simulink library "ammclib_bam_S32K3xx"  (R2016a)
(part 18 of 50)

      |   s16PropGainShift=ceil(log2(abs(fwkpf)));
      |   if s16PropGainShift<-31
      |     s16PropGainShift=-31;
      |   end
      |   if s16PropGainShift>31
      |     s16PropGainShift=31;
      |     warning(['Parameter s16PropGainShift of ' gcb ' exceeds the fixed-point range.']);
      |   end
      |   f32PropGain=round(fwkpf*2^(-s16PropGainShift)*2^31);
      |   if f32PropGain>2^31-1
      |     f32PropGain=2^31-1;
      |     warning(['Parameter f32PropGain of ' gcb ' exceeds the fixed-point range.']);
      |   end
      |   if f32PropGain<-2^31
      |     f32PropGain=-2^31;
      |     warning(['Parameter f32PropGain of ' gcb ' exceeds the fixed-point range.']);
      |   end
      |   s16IntegGainShift=ceil(log2(abs(kif)));
      |   if s16IntegGainShift<-31
      |     s16IntegGainShift=-31;
      |   end
      |   if s16IntegGainShift>31
      |     s16IntegGainShift=31;
      |     warning(['Parameter s16IntegGainShift of ' gcb ' exceeds the fixed-point range.']);
      |   end
      |   f32IntegGain=round(kif*2^(-s16IntegGainShift)*2^31);
      |   if f32IntegGain>2^31-1
      |     f32IntegGain=2^31-1;
      |     warning(['Parameter f32IntegGain of ' gcb ' exceeds the fixed-point range.']);
      |   end
      |   if f32IntegGain<-2^31
      |     f32IntegGain=-2^31;
      |     warning(['Parameter f32IntegGain of ' gcb ' exceeds the fixed-point range.']);
      |   end
      |   if (Idmax<0)
      |     iratio=abs(Idmax)/iscale;
      |     lowlim=0.3183098861837907*acos(iratio)-0.5;
      |   else
      |     lowlim=0.0;
      |   end
      |   f32LowerLimit=round(lowlim*2^31);
      |   if f32LowerLimit>2^31-1
      |     f32LowerLimit=2^31-1;
      |     warning(['Parameter f32LowerLimit of ' gcb ' exceeds the fixed-point range.']);
      |   end
      |   if f32LowerLimit<-2^31
      |     f32LowerLimit=-2^31;
      |     warning(['Parameter f32LowerLimit of ' gcb ' exceeds the fixed-point range.']);
      |   end
      |   f32UpperLimit=0;
      |   u16NSamples=round(log2(1.0/abs(lambdaFW)));
      |   if u16NSamples>31
      |     u16NSamples=31;
      |   end
      |   if u16NSamples<0
      |     u16NSamples=0;
      |   end
      |   if isnan(u16NSamples)
      |     if ~strcmp(u16NSamples_bkup,'0')
      |       set_param(gcb,'u16NSamples','0');
      |     end
      |   else
      |     tmps=num2str(u16NSamples);
      |     if ~strcmp(u16NSamples_bkup,tmps)
      |       set_param(gcb,'u16NSamples',tmps);
      |     end
      |   end
      |   if isnan(f32PropGain)
      |     if ~strcmp(f32PropGain_bkup,'0')
      |       set_param(gcb,'f32PropGain','0');
      |     end
      |   else
      |     tmps=num2str(f32PropGain);
      |     if ~strcmp(f32PropGain_bkup,tmps)
      |       set_param(gcb,'f32PropGain',tmps);
      |     end
      |   end
      |   if isnan(f32IntegGain)
      |     if ~strcmp(f32IntegGain_bkup,'0')
      |       set_param(gcb,'f32IntegGain','0');
      |     end
      |   else
      |     tmps=num2str(f32IntegGain);
      |     if ~strcmp(f32IntegGain_bkup,tmps)
      |       set_param(gcb,'f32IntegGain',tmps);
      |     end
      |   end
      |   if isnan(s16PropGainShift)
      |     if ~strcmp(s16PropGainShift_bkup,'0')
      |       set_param(gcb,'s16PropGainShift','0');
      |     end
      |   else
      |     tmps=num2str(s16PropGainShift);
      |     if ~strcmp(s16PropGainShift_bkup,tmps)
      |       set_param(gcb,'s16PropGainShift',tmps);
      |     end
      |   end
      |   if isnan(s16IntegGainShift)
      |     if ~strcmp(s16IntegGainShift_bkup,'0')
      |       set_param(gcb,'s16IntegGainShift','0');
      |     end
      |   else
      |     tmps=num2str(s16IntegGainShift);
      |     if ~strcmp(s16IntegGainShift_bkup,tmps)
      |       set_param(gcb,'s16IntegGainShift',tmps);
      |     end
      |   end
      |   if isnan(f32LowerLimit)
      |     if ~strcmp(f32LowerLimit_bkup,'0')
      |       set_param(gcb,'f32LowerLimit','0');
      |     end
      |   else
      |     tmps=num2str(f32LowerLimit);
      |     if ~strcmp(f32LowerLimit_bkup,tmps)
      |       set_param(gcb,'f32LowerLimit',tmps);
      |     end
      |   end
      |   if isnan(f32UpperLimit)
      |     if ~strcmp(f32UpperLimit_bkup,'0')
      |       set_param(gcb,'f32UpperLimit','0');
      |     end
      |   else
      |     tmps=num2str(f32UpperLimit);
      |     if ~strcmp(f32UpperLimit_bkup,tmps)
      |       set_param(gcb,'f32UpperLimit',tmps);
      |     end
      |   end
      | end
      mask Callback polepairs:
      | autoCalcEn=get_param(gcb,'autoCalcEn');
      | if strcmp(autoCalcEn,'on')
      |   SampleTime=Simulink.data.evalinGlobal(bdroot,get_param(gcb,'SampleTime'));
      |   if (SampleTime==-1)
      |     SampleTime=str2double(get_param(gcb,'SampleTime_1'));
      |   end
      |   u16NSamples_bkup=get_param(gcb,'u16NSamples');
      |   f32PropGain_bkup=get_param(gcb,'f32PropGain');
      |   f32IntegGain_bkup=get_param(gcb,'f32IntegGain');
      |   s16PropGainShift_bkup=get_param(gcb,'s16PropGainShift');
      |   s16IntegGainShift_bkup=get_param(gcb,'s16IntegGainShift');
      |   f32LowerLimit_bkup=get_param(gcb,'f32LowerLimit');
      |   f32UpperLimit_bkup=get_param(gcb,'f32UpperLimit');
      |   wf0=Simulink.data.evalinGlobal(bdroot,get_param(gcb,'wf0'));
      |   wksi=Simulink.data.evalinGlobal(bdroot,get_param(gcb,'wksi'));
      |   J=Simulink.data.evalinGlobal(bdroot,get_param(gcb,'J'));
      |   Kt=Simulink.data.evalinGlobal(bdroot,get_param(gcb,'Kt'));
      |   lambdaFW=Simulink.data.evalinGlobal(bdroot,get_param(gcb,'lambdaFW'));
      |   Idmax=Simulink.data.evalinGlobal(bdroot,get_param(gcb,'Idmax'));
      |   mechspeed=Simulink.data.evalinGlobal(bdroot,get_param(gcb,'mechspeed'));
      |   polepairs=Simulink.data.evalinGlobal(bdroot,get_param(gcb,'polepairs'));
      |   uscale=Simulink.data.evalinGlobal(bdroot,get_param(gcb,'uscale'));
      |   iscale=Simulink.data.evalinGlobal(bdroot,get_param(gcb,'iscale'));
      |   if (wf0<=0)
      |     warning('Natural frequency f0 must be positive.');
      |   end
      |   if (wksi<=0)
      |     warning('Current loop attenuation must be positive.');
      |   end
      |   if (wksi>1)
      |     warning('Current loop attenuation must not exceed 1.');
      |   end
      |   if (J<=0)
      |     warning('Moment of inertia J must be positive.');
      |   end
      |   if (Kt<=0)
      |     warning('Torque constant Kt must be positive.');
      |   end
      |   if (lambdaFW<0)
      |     warning('MA filter smoothing factor must be in the range 0..1.');
      |   end
      |   if (lambdaFW>1)
      |     warning('MA filter smoothing factor must be in the range 0..1.');
      |   end
      |   if (mechspeed<=0)
      |     warning('Max. speed must be positive.');
      |   end
      |   if (polepairs<1)
      |     warning('Number of pole pairs must be a natural number (1, 2, 3, ...).');
      |   end
      |   if (round(polepairs)~=polepairs)
      |     warning('Number of pole pairs must be a natural number (1, 2, 3, ...).');
      |   end
      |   if (uscale<=0)
      |     warning('U_max must be positive.');
      |   end
      |   if (iscale<=0)
      |     warning('I_max must be positive.');
      |   end
      |   w0=6.283185307179586*wf0;
      |   pgain=2.0*wksi*w0*J/Kt;
      |   igain=w0*w0*J/Kt;
      |   wmax=polepairs*mechspeed*0.1047197551196598;
      |   kif=igain*SampleTime*0.5*wmax/iscale;
      |   fwkpf=0.9*pgain*wmax/iscale;
      |   s16PropGainShift=ceil(log2(abs(fwkpf)));
      |   if s16PropGainShift<-31
      |     s16PropGainShift=-31;
      |   end
      |   if s16PropGainShift>31
      |     s16PropGainShift=31;
      |     warning(['Parameter s16PropGainShift of ' gcb ' exceeds the fixed-point range.']);
      |   end
      |   f32PropGain=round(fwkpf*2^(-s16PropGainShift)*2^31);
      |   if f32PropGain>2^31-1
      |     f32PropGain=2^31-1;
      |     warning(['Parameter f32PropGain of ' gcb ' exceeds the fixed-point range.']);
      |   end
      |   if f32PropGain<-2^31
      |     f32PropGain=-2^31;
      |     warning(['Parameter f32PropGain of ' gcb ' exceeds the fixed-point range.']);
      |   end
      |   s16IntegGainShift=ceil(log2(abs(kif)));
      |   if s16IntegGainShift<-31
      |     s16IntegGainShift=-31;
      |   end
      |   if s16IntegGainShift>31
      |     s16IntegGainShift=31;
      |     warning(['Parameter s16IntegGainShift of ' gcb ' exceeds the fixed-point range.']);
      |   end
      |   f32IntegGain=round(kif*2^(-s16IntegGainShift)*2^31);
      |   if f32IntegGain>2^31-1
      |     f32IntegGain=2^31-1;
      |     warning(['Parameter f32IntegGain of ' gcb ' exceeds the fixed-point range.']);
      |   end
      |   if f32IntegGain<-2^31
      |     f32IntegGain=-2^31;
      |     warning(['Parameter f32IntegGain of ' gcb ' exceeds the fixed-point range.']);
      |   end
      |   if (Idmax<0)
      |     iratio=abs(Idmax)/iscale;
      |     lowlim=0.3183098861837907*acos(iratio)-0.5;
      |   else
      |     lowlim=0.0;
      |   end
      |   f32LowerLimit=round(lowlim*2^31);
      |   if f32LowerLimit>2^31-1
      |     f32LowerLimit=2^31-1;
      |     warning(['Parameter f32LowerLimit of ' gcb ' exceeds the fixed-point range.']);
      |   end
      |   if f32LowerLimit<-2^31
      |     f32LowerLimit=-2^31;
      |     warning(['Parameter f32LowerLimit of ' gcb ' exceeds the fixed-point range.']);
      |   end
      |   f32UpperLimit=0;
      |   u16NSamples=round(log2(1.0/abs(lambdaFW)));
      |   if u16NSamples>31
      |     u16NSamples=31;
      |   end
      |   if u16NSamples<0
      |     u16NSamples=0;
      |   end
      |   if isnan(u16NSamples)
      |     if ~strcmp(u16NSamples_bkup,'0')
      |       set_param(gcb,'u16NSamples','0');
      |     end
      |   else
      |     tmps=num2str(u16NSamples);
      |     if ~strcmp(u16NSamples_bkup,tmps)
      |       set_param(gcb,'u16NSamples',tmps);
      |     end
      |   end
      |   if isnan(f32PropGain)
      |     if ~strcmp(f32PropGain_bkup,'0')
      |       set_param(gcb,'f32PropGain','0');
      |     end
      |   else
      |     tmps=num2str(f32PropGain);
      |     if ~strcmp(f32PropGain_bkup,tmps)
      |       set_param(gcb,'f32PropGain',tmps);
      |     end
      |   end
      |   if isnan(f32IntegGain)
      |     if ~strcmp(f32IntegGain_bkup,'0')
      |       set_param(gcb,'f32IntegGain','0');
      |     end
      |   else
      |     tmps=num2str(f32IntegGain);
      |     if ~strcmp(f32IntegGain_bkup,tmps)
      |       set_param(gcb,'f32IntegGain',tmps);
      |     end
      |   end
      |   if isnan(s16PropGainShift)
      |     if ~strcmp(s16PropGainShift_bkup,'0')
      |       set_param(gcb,'s16PropGainShift','0');
      |     end
      |   else
      |     tmps=num2str(s16PropGainShift);
      |     if ~strcmp(s16PropGainShift_bkup,tmps)
      |       set_param(gcb,'s16PropGainShift',tmps);
      |     end
      |   end
      |   if isnan(s16IntegGainShift)
      |     if ~strcmp(s16IntegGainShift_bkup,'0')
      |       set_param(gcb,'s16IntegGainShift','0');
      |     end
      |   else
      |     tmps=num2str(s16IntegGainShift);
      |     if ~strcmp(s16IntegGainShift_bkup,tmps)
      |       set_param(gcb,'s16IntegGainShift',tmps);
      |     end
      |   end
      |   if isnan(f32LowerLimit)
      |     if ~strcmp(f32LowerLimit_bkup,'0')
      |       set_param(gcb,'f32LowerLimit','0');
      |     end
      |   else
      |     tmps=num2str(f32LowerLimit);
      |     if ~strcmp(f32LowerLimit_bkup,tmps)
      |       set_param(gcb,'f32LowerLimit',tmps);
      |     end
      |   end
      |   if isnan(f32UpperLimit)
      |     if ~strcmp(f32UpperLimit_bkup,'0')
      |       set_param(gcb,'f32UpperLimit','0');
      |     end
      |   else
      |     tmps=num2str(f32UpperLimit);
      |     if ~strcmp(f32UpperLimit_bkup,tmps)
      |       set_param(gcb,'f32UpperLimit',tmps);
      |     end
      |   end
      | end
      mask Callback uscale:
      | autoCalcEn=get_param(gcb,'autoCalcEn');
      | if strcmp(autoCalcEn,'on')
      |   SampleTime=Simulink.data.evalinGlobal(bdroot,get_param(gcb,'SampleTime'));
      |   if (SampleTime==-1)
      |     SampleTime=str2double(get_param(gcb,'SampleTime_1'));
      |   end
      |   u16NSamples_bkup=get_param(gcb,'u16NSamples');
      |   f32PropGain_bkup=get_param(gcb,'f32PropGain');
      |   f32IntegGain_bkup=get_param(gcb,'f32IntegGain');
      |   s16PropGainShift_bkup=get_param(gcb,'s16PropGainShift');
      |   s16IntegGainShift_bkup=get_param(gcb,'s16IntegGainShift');
      |   f32LowerLimit_bkup=get_param(gcb,'f32LowerLimit');
      |   f32UpperLimit_bkup=get_param(gcb,'f32UpperLimit');
      |   wf0=Simulink.data.evalinGlobal(bdroot,get_param(gcb,'wf0'));
      |   wksi=Simulink.data.evalinGlobal(bdroot,get_param(gcb,'wksi'));
      |   J=Simulink.data.evalinGlobal(bdroot,get_param(gcb,'J'));
      |   Kt=Simulink.data.evalinGlobal(bdroot,get_param(gcb,'Kt'));
      |   lambdaFW=Simulink.data.evalinGlobal(bdroot,get_param(gcb,'lambdaFW'));
      |   Idmax=Simulink.data.evalinGlobal(bdroot,get_param(gcb,'Idmax'));
      |   mechspeed=Simulink.data.evalinGlobal(bdroot,get_param(gcb,'mechspeed'));
      |   polepairs=Simulink.data.evalinGlobal(bdroot,get_param(gcb,'polepairs'));
      |   uscale=Simulink.data.evalinGlobal(bdroot,get_param(gcb,'uscale'));
      |   iscale=Simulink.data.evalinGlobal(bdroot,get_param(gcb,'iscale'));
      |   if (wf0<=0)
      |     warning('Natural frequency f0 must be positive.');
      |   end
      |   if (wksi<=0)
      |     warning('Current loop attenuation must be positive.');
      |   end
      |   if (wksi>1)
      |     warning('Current loop attenuation must not exceed 1.');
      |   end
      |   if (J<=0)
      |     warning('Moment of inertia J must be positive.');
      |   end
      |   if (Kt<=0)
      |     warning('Torque constant Kt must be positive.');
      |   end
      |   if (lambdaFW<0)
      |     warning('MA filter smoothing factor must be in the range 0..1.');
      |   end
      |   if (lambdaFW>1)
      |     warning('MA filter smoothing factor must be in the range 0..1.');
      |   end
      |   if (mechspeed<=0)
      |     warning('Max. speed must be positive.');
      |   end
      |   if (polepairs<1)
      |     warning('Number of pole pairs must be a natural number (1, 2, 3, ...).');
      |   end
      |   if (round(polepairs)~=polepairs)
      |     warning('Number of pole pairs must be a natural number (1, 2, 3, ...).');
      |   end
      |   if (uscale<=0)
      |     warning('U_max must be positive.');
      |   end
      |   if (iscale<=0)
      |     warning('I_max must be positive.');
      |   end
      |   w0=6.283185307179586*wf0;
      |   pgain=2.0*wksi*w0*J/Kt;
      |   igain=w0*w0*J/Kt;
      |   wmax=polepairs*mechspeed*0.1047197551196598;
      |   kif=igain*SampleTime*0.5*wmax/iscale;
      |   fwkpf=0.9*pgain*wmax/iscale;
      |   s16PropGainShift=ceil(log2(abs(fwkpf)));
      |   if s16PropGainShift<-31
      |     s16PropGainShift=-31;
      |   end
      |   if s16PropGainShift>31
      |     s16PropGainShift=31;
      |     warning(['Parameter s16PropGainShift of ' gcb ' exceeds the fixed-point range.']);
      |   end
      |   f32PropGain=round(fwkpf*2^(-s16PropGainShift)*2^31);
      |   if f32PropGain>2^31-1
      |     f32PropGain=2^31-1;
      |     warning(['Parameter f32PropGain of ' gcb ' exceeds the fixed-point range.']);
      |   end
      |   if f32PropGain<-2^31
      |     f32PropGain=-2^31;
      |     warning(['Parameter f32PropGain of ' gcb ' exceeds the fixed-point range.']);
      |   end
      |   s16IntegGainShift=ceil(log2(abs(kif)));
      |   if s16IntegGainShift<-31
      |     s16IntegGainShift=-31;
      |   end
      |   if s16IntegGainShift>31
      |     s16IntegGainShift=31;
      |     warning(['Parameter s16IntegGainShift of ' gcb ' exceeds the fixed-point range.']);
      |   end
      |   f32IntegGain=round(kif*2^(-s16IntegGainShift)*2^31);
      |   if f32IntegGain>2^31-1
      |     f32IntegGain=2^31-1;
      |     warning(['Parameter f32IntegGain of ' gcb ' exceeds the fixed-point range.']);
      |   end
      |   if f32IntegGain<-2^31
      |     f32IntegGain=-2^31;
      |     warning(['Parameter f32IntegGain of ' gcb ' exceeds the fixed-point range.']);
      |   end
      |   if (Idmax<0)
      |     iratio=abs(Idmax)/iscale;
      |     lowlim=0.3183098861837907*acos(iratio)-0.5;
      |   else
      |     lowlim=0.0;
      |   end
      |   f32LowerLimit=round(lowlim*2^31);
      |   if f32LowerLimit>2^31-1
      |     f32LowerLimit=2^31-1;
      |     warning(['Parameter f32LowerLimit of ' gcb ' exceeds the fixed-point range.']);
      |   end
      |   if f32LowerLimit<-2^31
      |     f32LowerLimit=-2^31;
      |     warning(['Parameter f32LowerLimit of ' gcb ' exceeds the fixed-point range.']);
      |   end
      |   f32UpperLimit=0;
      |   u16NSamples=round(log2(1.0/abs(lambdaFW)));
      |   if u16NSamples>31
      |     u16NSamples=31;
      |   end
      |   if u16NSamples<0
      |     u16NSamples=0;
      |   end
      |   if isnan(u16NSamples)
      |     if ~strcmp(u16NSamples_bkup,'0')
      |       set_param(gcb,'u16NSamples','0');
      |     end
      |   else
      |     tmps=num2str(u16NSamples);
      |     if ~strcmp(u16NSamples_bkup,tmps)
      |       set_param(gcb,'u16NSamples',tmps);
      |     end
      |   end
      |   if isnan(f32PropGain)
      |     if ~strcmp(f32PropGain_bkup,'0')
      |       set_param(gcb,'f32PropGain','0');
      |     end
      |   else
      |     tmps=num2str(f32PropGain);
      |     if ~strcmp(f32PropGain_bkup,tmps)
      |       set_param(gcb,'f32PropGain',tmps);
      |     end
      |   end
      |   if isnan(f32IntegGain)
      |     if ~strcmp(f32IntegGain_bkup,'0')
      |       set_param(gcb,'f32IntegGain','0');
      |     end
      |   else
      |     tmps=num2str(f32IntegGain);
      |     if ~strcmp(f32IntegGain_bkup,tmps)
      |       set_param(gcb,'f32IntegGain',tmps);
      |     end
      |   end
      |   if isnan(s16PropGainShift)
      |     if ~strcmp(s16PropGainShift_bkup,'0')
      |       set_param(gcb,'s16PropGainShift','0');
      |     end
      |   else
      |     tmps=num2str(s16PropGainShift);
      |     if ~strcmp(s16PropGainShift_bkup,tmps)
      |       set_param(gcb,'s16PropGainShift',tmps);
      |     end
      |   end
      |   if isnan(s16IntegGainShift)
      |     if ~strcmp(s16IntegGainShift_bkup,'0')
      |       set_param(gcb,'s16IntegGainShift','0');
      |     end
      |   else
      |     tmps=num2str(s16IntegGainShift);
      |     if ~strcmp(s16IntegGainShift_bkup,tmps)
      |       set_param(gcb,'s16IntegGainShift',tmps);
      |     end
      |   end
      |   if isnan(f32LowerLimit)
      |     if ~strcmp(f32LowerLimit_bkup,'0')
      |       set_param(gcb,'f32LowerLimit','0');
      |     end
      |   else
      |     tmps=num2str(f32LowerLimit);
      |     if ~strcmp(f32LowerLimit_bkup,tmps)
      |       set_param(gcb,'f32LowerLimit',tmps);
      |     end
      |   end
      |   if isnan(f32UpperLimit)
      |     if ~strcmp(f32UpperLimit_bkup,'0')
      |       set_param(gcb,'f32UpperLimit','0');
      |     end
      |   else
      |     tmps=num2str(f32UpperLimit);
      |     if ~strcmp(f32UpperLimit_bkup,tmps)
      |       set_param(gcb,'f32UpperLimit',tmps);
      |     end
      |   end
      | end
      mask Callback iscale:
      | autoCalcEn=get_param(gcb,'autoCalcEn');
      | if strcmp(autoCalcEn,'on')
      |   SampleTime=Simulink.data.evalinGlobal(bdroot,get_param(gcb,'SampleTime'));
      |   if (SampleTime==-1)
      |     SampleTime=str2double(get_param(gcb,'SampleTime_1'));
      |   end
      |   u16NSamples_bkup=get_param(gcb,'u16NSamples');
      |   f32PropGain_bkup=get_param(gcb,'f32PropGain');
      |   f32IntegGain_bkup=get_param(gcb,'f32IntegGain');
      |   s16PropGainShift_bkup=get_param(gcb,'s16PropGainShift');
      |   s16IntegGainShift_bkup=get_param(gcb,'s16IntegGainShift');
      |   f32LowerLimit_bkup=get_param(gcb,'f32LowerLimit');
      |   f32UpperLimit_bkup=get_param(gcb,'f32UpperLimit');
      |   wf0=Simulink.data.evalinGlobal(bdroot,get_param(gcb,'wf0'));
      |   wksi=Simulink.data.evalinGlobal(bdroot,get_param(gcb,'wksi'));
      |   J=Simulink.data.evalinGlobal(bdroot,get_param(gcb,'J'));
      |   Kt=Simulink.data.evalinGlobal(bdroot,get_param(gcb,'Kt'));
      |   lambdaFW=Simulink.data.evalinGlobal(bdroot,get_param(gcb,'lambdaFW'));
      |   Idmax=Simulink.data.evalinGlobal(bdroot,get_param(gcb,'Idmax'));
      |   mechspeed=Simulink.data.evalinGlobal(bdroot,get_param(gcb,'mechspeed'));
      |   polepairs=Simulink.data.evalinGlobal(bdroot,get_param(gcb,'polepairs'));
      |   uscale=Simulink.data.evalinGlobal(bdroot,get_param(gcb,'uscale'));
      |   iscale=Simulink.data.evalinGlobal(bdroot,get_param(gcb,'iscale'));
      |   if (wf0<=0)
      |     warning('Natural frequency f0 must be positive.');
      |   end
      |   if (wksi<=0)
      |     warning('Current loop attenuation must be positive.');
      |   end
      |   if (wksi>1)
      |     warning('Current loop attenuation must not exceed 1.');
      |   end
      |   if (J<=0)
      |     warning('Moment of inertia J must be positive.');
      |   end
      |   if (Kt<=0)
      |     warning('Torque constant Kt must be positive.');
      |   end
      |   if (lambdaFW<0)
      |     warning('MA filter smoothing factor must be in the range 0..1.');
      |   end
      |   if (lambdaFW>1)
      |     warning('MA filter smoothing factor must be in the range 0..1.');
      |   end
      |   if (mechspeed<=0)
      |     warning('Max. speed must be positive.');
      |   end
      |   if (polepairs<1)
      |     warning('Number of pole pairs must be a natural number (1, 2, 3, ...).');
      |   end
      |   if (round(polepairs)~=polepairs)
      |     warning('Number of pole pairs must be a natural number (1, 2, 3, ...).');
      |   end
      |   if (uscale<=0)
      |     warning('U_max must be positive.');
      |   end
      |   if (iscale<=0)
      |     warning('I_max must be positive.');
      |   end
      |   w0=6.283185307179586*wf0;
      |   pgain=2.0*wksi*w0*J/Kt;
      |   igain=w0*w0*J/Kt;
      |   wmax=polepairs*mechspeed*0.1047197551196598;
      |   kif=igain*SampleTime*0.5*wmax/iscale;
      |   fwkpf=0.9*pgain*wmax/iscale;
      |   s16PropGainShift=ceil(log2(abs(fwkpf)));
      |   if s16PropGainShift<-31
      |     s16PropGainShift=-31;
      |   end
      |   if s16PropGainShift>31
      |     s16PropGainShift=31;
      |     warning(['Parameter s16PropGainShift of ' gcb ' exceeds the fixed-point range.']);
      |   end
      |   f32PropGain=round(fwkpf*2^(-s16PropGainShift)*2^31);
      |   if f32PropGain>2^31-1
      |     f32PropGain=2^31-1;
      |     warning(['Parameter f32PropGain of ' gcb ' exceeds the fixed-point range.']);
      |   end
      |   if f32PropGain<-2^31
      |     f32PropGain=-2^31;
      |     warning(['Parameter f32PropGain of ' gcb ' exceeds the fixed-point range.']);
      |   end
      |   s16IntegGainShift=ceil(log2(abs(kif)));
      |   if s16IntegGainShift<-31
      |     s16IntegGainShift=-31;
      |   end
      |   if s16IntegGainShift>31
      |     s16IntegGainShift=31;
      |     warning(['Parameter s16IntegGainShift of ' gcb ' exceeds the fixed-point range.']);
      |   end
      |   f32IntegGain=round(kif*2^(-s16IntegGainShift)*2^31);
      |   if f32IntegGain>2^31-1
      |     f32IntegGain=2^31-1;
      |     warning(['Parameter f32IntegGain of ' gcb ' exceeds the fixed-point range.']);
      |   end
      |   if f32IntegGain<-2^31
      |     f32IntegGain=-2^31;
      |     warning(['Parameter f32IntegGain of ' gcb ' exceeds the fixed-point range.']);
      |   end
      |   if (Idmax<0)
      |     iratio=abs(Idmax)/iscale;
      |     lowlim=0.3183098861837907*acos(iratio)-0.5;
      |   else
      |     lowlim=0.0;
      |   end
      |   f32LowerLimit=round(lowlim*2^31);
      |   if f32LowerLimit>2^31-1
      |     f32LowerLimit=2^31-1;
      |     warning(['Parameter f32LowerLimit of ' gcb ' exceeds the fixed-point range.']);
      |   end
      |   if f32LowerLimit<-2^31
      |     f32LowerLimit=-2^31;
      |     warning(['Parameter f32LowerLimit of ' gcb ' exceeds the fixed-point range.']);
      |   end
      |   f32UpperLimit=0;
      |   u16NSamples=round(log2(1.0/abs(lambdaFW)));
      |   if u16NSamples>31
      |     u16NSamples=31;
      |   end
      |   if u16NSamples<0
      |     u16NSamples=0;
      |   end
      |   if isnan(u16NSamples)
      |     if ~strcmp(u16NSamples_bkup,'0')
      |       set_param(gcb,'u16NSamples','0');
      |     end
      |   else
      |     tmps=num2str(u16NSamples);
      |     if ~strcmp(u16NSamples_bkup,tmps)
      |       set_param(gcb,'u16NSamples',tmps);
      |     end
      |   end
      |   if isnan(f32PropGain)
      |     if ~strcmp(f32PropGain_bkup,'0')
      |       set_param(gcb,'f32PropGain','0');
      |     end
      |   else
      |     tmps=num2str(f32PropGain);
      |     if ~strcmp(f32PropGain_bkup,tmps)
      |       set_param(gcb,'f32PropGain',tmps);
      |     end
      |   end
      |   if isnan(f32IntegGain)
      |     if ~strcmp(f32IntegGain_bkup,'0')
      |       set_param(gcb,'f32IntegGain','0');
      |     end
      |   else
      |     tmps=num2str(f32IntegGain);
      |     if ~strcmp(f32IntegGain_bkup,tmps)
      |       set_param(gcb,'f32IntegGain',tmps);
      |     end
      |   end
      |   if isnan(s16PropGainShift)
      |     if ~strcmp(s16PropGainShift_bkup,'0')
      |       set_param(gcb,'s16PropGainShift','0');
      |     end
      |   else
      |     tmps=num2str(s16PropGainShift);
      |     if ~strcmp(s16PropGainShift_bkup,tmps)
      |       set_param(gcb,'s16PropGainShift',tmps);
      |     end
      |   end
      |   if isnan(s16IntegGainShift)
      |     if ~strcmp(s16IntegGainShift_bkup,'0')
      |       set_param(gcb,'s16IntegGainShift','0');
      |     end
      |   else
      |     tmps=num2str(s16IntegGainShift);
      |     if ~strcmp(s16IntegGainShift_bkup,tmps)
      |       set_param(gcb,'s16IntegGainShift',tmps);
      |     end
      |   end
      |   if isnan(f32LowerLimit)
      |     if ~strcmp(f32LowerLimit_bkup,'0')
      |       set_param(gcb,'f32LowerLimit','0');
      |     end
      |   else
      |     tmps=num2str(f32LowerLimit);
      |     if ~strcmp(f32LowerLimit_bkup,tmps)
      |       set_param(gcb,'f32LowerLimit',tmps);
      |     end
      |   end
      |   if isnan(f32UpperLimit)
      |     if ~strcmp(f32UpperLimit_bkup,'0')
      |       set_param(gcb,'f32UpperLimit','0');
      |     end
      |   else
      |     tmps=num2str(f32UpperLimit);
      |     if ~strcmp(f32UpperLimit_bkup,tmps)
      |       set_param(gcb,'f32UpperLimit',tmps);
      |     end
      |   end
      | end
      mask Callback autoCalcEn:
      | maskStr=get_param(gcb,'showStates');
      | if strcmp(maskStr,'Hide (faster execution)')
      |   p=Simulink.Mask.get(gcb);
      |   autoCalcEn=get_param(gcb,'autoCalcEn');
      |   hintText=p.getDialogControl('timeHint');
      |   if strcmp(autoCalcEn,'on')
      |     param=p.getParameter('iscale');
      |     if strcmp(param.Enabled,'off')
      |       SampleTime=Simulink.data.evalinGlobal(bdroot,get_param(gcb,'SampleTime'));
      |       if SampleTime==-1
      |         SampleTime=str2double(get_param(gcb,'SampleTime_1'));
      |         if isnan(SampleTime)
      |           hintText.Prompt=['Note: Implementation parameters cannot be calculated yet because the block''s inherited sample time is unknown. Simulink will update the sample time when you run the simulation.'];
      |         else
      |           hintText.Prompt=['Caution: Implementation parameters depend on inherited sample time. Make sure that the sample time of the block''s inputs corresponds to the sampling period in the target application.'];
      |         end
      |       else
      |         hintText.Prompt='Caution: Implementation parameters depend on the sample time. Make sure that the simulation time step corresponds to the sampling period in the target application.';
      |       end
      |       p=Simulink.Mask.get(gcb);
      |       param=p.getParameter('wf0');
      |       param.set('Enabled','on');
      |       param=p.getParameter('wksi');
      |       param.set('Enabled','on');
      |       param=p.getParameter('J');
      |       param.set('Enabled','on');
      |       param=p.getParameter('Kt');
      |       param.set('Enabled','on');
      |       param=p.getParameter('lambdaFW');
      |       param.set('Enabled','on');
      |       param=p.getParameter('Idmax');
      |       param.set('Enabled','on');
      |       param=p.getParameter('mechspeed');
      |       param.set('Enabled','on');
      |       param=p.getParameter('polepairs');
      |       param.set('Enabled','on');
      |       param=p.getParameter('uscale');
      |       param.set('Enabled','on');
      |       param=p.getParameter('iscale');
      |       param.set('Enabled','on');
      |     else
      |       SampleTime=Simulink.data.evalinGlobal(bdroot,get_param(gcb,'SampleTime'));
      |       if SampleTime==-1
      |         SampleTime=str2double(get_param(gcb,'SampleTime_1'));
      |       end
      |     end
      |     u16NSamples_bkup=get_param(gcb,'u16NSamples');
      |     f32PropGain_bkup=get_param(gcb,'f32PropGain');
      |     f32IntegGain_bkup=get_param(gcb,'f32IntegGain');
      |     s16PropGainShift_bkup=get_param(gcb,'s16PropGainShift');
      |     s16IntegGainShift_bkup=get_param(gcb,'s16IntegGainShift');
      |     f32LowerLimit_bkup=get_param(gcb,'f32LowerLimit');
      |     f32UpperLimit_bkup=get_param(gcb,'f32UpperLimit');
      |     wf0=Simulink.data.evalinGlobal(bdroot,get_param(gcb,'wf0'));
      |     wksi=Simulink.data.evalinGlobal(bdroot,get_param(gcb,'wksi'));
      |     J=Simulink.data.evalinGlobal(bdroot,get_param(gcb,'J'));
      |     Kt=Simulink.data.evalinGlobal(bdroot,get_param(gcb,'Kt'));
      |     lambdaFW=Simulink.data.evalinGlobal(bdroot,get_param(gcb,'lambdaFW'));
      |     Idmax=Simulink.data.evalinGlobal(bdroot,get_param(gcb,'Idmax'));
      |     mechspeed=Simulink.data.evalinGlobal(bdroot,get_param(gcb,'mechspeed'));
      |     polepairs=Simulink.data.evalinGlobal(bdroot,get_param(gcb,'polepairs'));
      |     uscale=Simulink.data.evalinGlobal(bdroot,get_param(gcb,'uscale'));
      |     iscale=Simulink.data.evalinGlobal(bdroot,get_param(gcb,'iscale'));
      |     if (wf0<=0)
      |       warning('Natural frequency f0 must be positive.');
      |     end
      |     if (wksi<=0)
      |       warning('Current loop attenuation must be positive.');
      |     end
      |     if (wksi>1)
      |       warning('Current loop attenuation must not exceed 1.');
      |     end
      |     if (J<=0)
      |       warning('Moment of inertia J must be positive.');
      |     end
      |     if (Kt<=0)
      |       warning('Torque constant Kt must be positive.');
      |     end
      |     if (lambdaFW<0)
      |       warning('MA filter smoothing factor must be in the range 0..1.');
      |     end
      |     if (lambdaFW>1)
      |       warning('MA filter smoothing factor must be in the range 0..1.');
      |     end
      |     if (mechspeed<=0)
      |       warning('Max. speed must be positive.');
      |     end
      |     if (polepairs<1)
      |       warning('Number of pole pairs must be a natural number (1, 2, 3, ...).');
      |     end
      |     if (round(polepairs)~=polepairs)
      |       warning('Number of pole pairs must be a natural number (1, 2, 3, ...).');
      |     end
      |     if (uscale<=0)
      |       warning('U_max must be positive.');
      |     end
      |     if (iscale<=0)
      |       warning('I_max must be positive.');
      |     end
      |     w0=6.283185307179586*wf0;
      |     pgain=2.0*wksi*w0*J/Kt;
      |     igain=w0*w0*J/Kt;
      |     wmax=polepairs*mechspeed*0.1047197551196598;
      |     kif=igain*SampleTime*0.5*wmax/iscale;
      |     fwkpf=0.9*pgain*wmax/iscale;
      |     s16PropGainShift=ceil(log2(abs(fwkpf)));
      |     if s16PropGainShift<-31
      |       s16PropGainShift=-31;
      |     end
      |     if s16PropGainShift>31
      |       s16PropGainShift=31;
      |       warning(['Parameter s16PropGainShift of ' gcb ' exceeds the fixed-point range.']);
      |     end
      |     f32PropGain=round(fwkpf*2^(-s16PropGainShift)*2^31);
      |     if f32PropGain>2^31-1
      |       f32PropGain=2^31-1;
      |       warning(['Parameter f32PropGain of ' gcb ' exceeds the fixed-point range.']);
      |     end
      |     if f32PropGain<-2^31
      |       f32PropGain=-2^31;
      |       warning(['Parameter f32PropGain of ' gcb ' exceeds the fixed-point range.']);
      |     end
      |     s16IntegGainShift=ceil(log2(abs(kif)));
      |     if s16IntegGainShift<-31
      |       s16IntegGainShift=-31;
      |     end
      |     if s16IntegGainShift>31
      |       s16IntegGainShift=31;
      |       warning(['Parameter s16IntegGainShift of ' gcb ' exceeds the fixed-point range.']);
      |     end
      |     f32IntegGain=round(kif*2^(-s16IntegGainShift)*2^31);
      |     if f32IntegGain>2^31-1
      |       f32IntegGain=2^31-1;
      |       warning(['Parameter f32IntegGain of ' gcb ' exceeds the fixed-point range.']);
      |     end
      |     if f32IntegGain<-2^31
      |       f32IntegGain=-2^31;
      |       warning(['Parameter f32IntegGain of ' gcb ' exceeds the fixed-point range.']);
      |     end
      |     if (Idmax<0)
      |       iratio=abs(Idmax)/iscale;
      |       lowlim=0.3183098861837907*acos(iratio)-0.5;
      |     else
      |       lowlim=0.0;
      |     end
      |     f32LowerLimit=round(lowlim*2^31);
      |     if f32LowerLimit>2^31-1
      |       f32LowerLimit=2^31-1;
      |       warning(['Parameter f32LowerLimit of ' gcb ' exceeds the fixed-point range.']);
      |     end
      |     if f32LowerLimit<-2^31
      |       f32LowerLimit=-2^31;
      |       warning(['Parameter f32LowerLimit of ' gcb ' exceeds the fixed-point range.']);
      |     end
      |     f32UpperLimit=0;
      |     u16NSamples=round(log2(1.0/abs(lambdaFW)));
      |     if u16NSamples>31
      |       u16NSamples=31;
      |     end
      |     if u16NSamples<0
      |       u16NSamples=0;
      |     end
      |     if isnan(u16NSamples)
      |       if ~strcmp(u16NSamples_bkup,'0')
      |         set_param(gcb,'u16NSamples','0');
      |       end
      |     else
      |       tmps=num2str(u16NSamples);
      |       if ~strcmp(u16NSamples_bkup,tmps)
      |         set_param(gcb,'u16NSamples',tmps);
      |       end
      |     end
      |     if isnan(f32PropGain)
      |       if ~strcmp(f32PropGain_bkup,'0')
      |         set_param(gcb,'f32PropGain','0');
      |       end
      |     else
      |       tmps=num2str(f32PropGain);
      |       if ~strcmp(f32PropGain_bkup,tmps)
      |         set_param(gcb,'f32PropGain',tmps);
      |       end
      |     end
      |     if isnan(f32IntegGain)
      |       if ~strcmp(f32IntegGain_bkup,'0')
      |         set_param(gcb,'f32IntegGain','0');
      |       end
      |     else
      |       tmps=num2str(f32IntegGain);
      |       if ~strcmp(f32IntegGain_bkup,tmps)
      |         set_param(gcb,'f32IntegGain',tmps);
      |       end
      |     end
      |     if isnan(s16PropGainShift)
      |       if ~strcmp(s16PropGainShift_bkup,'0')
      |         set_param(gcb,'s16PropGainShift','0');
      |       end
      |     else
      |       tmps=num2str(s16PropGainShift);
      |       if ~strcmp(s16PropGainShift_bkup,tmps)
      |         set_param(gcb,'s16PropGainShift',tmps);
      |       end
      |     end
      |     if isnan(s16IntegGainShift)
      |       if ~strcmp(s16IntegGainShift_bkup,'0')
      |         set_param(gcb,'s16IntegGainShift','0');
      |       end
      |     else
      |       tmps=num2str(s16IntegGainShift);
      |       if ~strcmp(s16IntegGainShift_bkup,tmps)
      |         set_param(gcb,'s16IntegGainShift',tmps);
      |       end
      |     end
      |     if isnan(f32LowerLimit)
      |       if ~strcmp(f32LowerLimit_bkup,'0')
      |         set_param(gcb,'f32LowerLimit','0');
      |       end
      |     else
      |       tmps=num2str(f32LowerLimit);
      |       if ~strcmp(f32LowerLimit_bkup,tmps)
      |         set_param(gcb,'f32LowerLimit',tmps);
      |       end
      |     end
      |     if isnan(f32UpperLimit)
      |       if ~strcmp(f32UpperLimit_bkup,'0')
      |         set_param(gcb,'f32UpperLimit','0');
      |       end
      |     else
      |       tmps=num2str(f32UpperLimit);
      |       if ~strcmp(f32UpperLimit_bkup,tmps)
      |         set_param(gcb,'f32UpperLimit',tmps);
      |       end
      |     end
      |   else
      |     param=p.getParameter('iscale');
      |     if strcmp(param.Enabled,'on')
      |       hintText.Prompt='Caution: Implementation parameters are fixed.';
      |       p=Simulink.Mask.get(gcb);
      |       param=p.getParameter('wf0');
      |       param.set('Enabled','off');
      |       param=p.getParameter('wksi');
      |       param.set('Enabled','off');
      |       param=p.getParameter('J');
      |       param.set('Enabled','off');
      |       param=p.getParameter('Kt');
      |       param.set('Enabled','off');
      |       param=p.getParameter('lambdaFW');
      |       param.set('Enabled','off');
      |       param=p.getParameter('Idmax');
      |       param.set('Enabled','off');
      |       param=p.getParameter('mechspeed');
      |       param.set('Enabled','off');
      |       param=p.getParameter('polepairs');
      |       param.set('Enabled','off');
      |       param=p.getParameter('uscale');
      |       param.set('Enabled','off');
      |       param=p.getParameter('iscale');
      |       param.set('Enabled','off');
      |     end
      |   end
      | end
      mask DialogControl CompBut Prompt: Recalculate sample times
      mask DialogControl CompBut Tooltip: Simulink updates the sample times of all blocks when the simulation is run. This button will update the sample times now.
      mask DialogControl CompBut Callback:
      | btn=questdlg('This will apply all changes in all open dialog boxes and update the schematic. Do you want to proceed?','Apply all changes','Continue','Cancel','Continue');
      | if strcmp(btn,'Continue')
      |   dlgs=DAStudio.ToolRoot.getOpenDialogs;
      |   for i=1:length(dlgs)
      |     dlgs(i).apply;
      |   end
      |   try
      |     SampleTime_1=str2double(get_param(gcb,'SampleTime_1'));
      |     ts=Simulink.Block.getSampleTimes(gcb);
      |     ts=ts(1).Value(1);
      |     if (SampleTime_1 ~= ts)
      |       SampleTime_1=ts;
      |       set_param(gcb,'SampleTime_1',num2str(ts));
      |       autoCalcEn=get_param(gcb,'autoCalcEn');
      |       if strcmp(autoCalcEn,'on')
      |         SampleTime=Simulink.data.evalinGlobal(bdroot,get_param(gcb,'SampleTime'));
      |         p=Simulink.Mask.get(gcb);
      |         hintText=p.getDialogControl('timeHint');
      |         if SampleTime==-1
      |           SampleTime=SampleTime_1;
      |           hintText.Prompt='Caution: Implementation parameters depend on inherited sample time. Make sure that the sample time of the block''s inputs corresponds to the sampling period in the target application.';
      |         else
      |           hintText.Prompt='Caution: Implementation parameters depend on the sample time. Make sure that the simulation time step corresponds to the sampling period in the target application.';
      |         end
      |         u16NSamples_bkup=get_param(gcb,'u16NSamples');
      |         f32PropGain_bkup=get_param(gcb,'f32PropGain');
      |         f32IntegGain_bkup=get_param(gcb,'f32IntegGain');
      |         s16PropGainShift_bkup=get_param(gcb,'s16PropGainShift');
      |         s16IntegGainShift_bkup=get_param(gcb,'s16IntegGainShift');
      |         f32LowerLimit_bkup=get_param(gcb,'f32LowerLimit');
      |         f32UpperLimit_bkup=get_param(gcb,'f32UpperLimit');
      |         wf0=Simulink.data.evalinGlobal(bdroot,get_param(gcb,'wf0'));
      |         wksi=Simulink.data.evalinGlobal(bdroot,get_param(gcb,'wksi'));
      |         J=Simulink.data.evalinGlobal(bdroot,get_param(gcb,'J'));
      |         Kt=Simulink.data.evalinGlobal(bdroot,get_param(gcb,'Kt'));
      |         lambdaFW=Simulink.data.evalinGlobal(bdroot,get_param(gcb,'lambdaFW'));
      |         Idmax=Simulink.data.evalinGlobal(bdroot,get_param(gcb,'Idmax'));
      |         mechspeed=Simulink.data.evalinGlobal(bdroot,get_param(gcb,'mechspeed'));
      |         polepairs=Simulink.data.evalinGlobal(bdroot,get_param(gcb,'polepairs'));
      |         uscale=Simulink.data.evalinGlobal(bdroot,get_param(gcb,'uscale'));
      |         iscale=Simulink.data.evalinGlobal(bdroot,get_param(gcb,'iscale'));
      |         if (wf0<=0)
      |           warning('Natural frequency f0 must be positive.');
      |         end
      |         if (wksi<=0)
      |           warning('Current loop attenuation must be positive.');
      |         end
      |         if (wksi>1)
      |           warning('Current loop attenuation must not exceed 1.');
      |         end
      |         if (J<=0)
      |           warning('Moment of inertia J must be positive.');
      |         end
      |         if (Kt<=0)
      |           warning('Torque constant Kt must be positive.');
      |         end
      |         if (lambdaFW<0)
      |           warning('MA filter smoothing factor must be in the range 0..1.');
      |         end
      |         if (lambdaFW>1)
      |           warning('MA filter smoothing factor must be in the range 0..1.');
      |         end
      |         if (mechspeed<=0)
      |           warning('Max. speed must be positive.');
      |         end
      |         if (polepairs<1)
      |           warning('Number of pole pairs must be a natural number (1, 2, 3, ...).');
      |         end
      |         if (round(polepairs)~=polepairs)
      |           warning('Number of pole pairs must be a natural number (1, 2, 3, ...).');
      |         end
      |         if (uscale<=0)
      |           warning('U_max must be positive.');
      |         end
      |         if (iscale<=0)
      |           warning('I_max must be positive.');
      |         end
      |         w0=6.283185307179586*wf0;
      |         pgain=2.0*wksi*w0*J/Kt;
      |         igain=w0*w0*J/Kt;
      |         wmax=polepairs*mechspeed*0.1047197551196598;
      |         kif=igain*SampleTime*0.5*wmax/iscale;
      |         fwkpf=0.9*pgain*wmax/iscale;
      |         s16PropGainShift=ceil(log2(abs(fwkpf)));
      |         if s16PropGainShift<-31
      |           s16PropGainShift=-31;
      |         end
      |         if s16PropGainShift>31
      |           s16PropGainShift=31;
      |           warning(['Parameter s16PropGainShift of ' gcb ' exceeds the fixed-point range.']);
      |         end
      |         f32PropGain=round(fwkpf*2^(-s16PropGainShift)*2^31);
      |         if f32PropGain>2^31-1
      |           f32PropGain=2^31-1;
      |           warning(['Parameter f32PropGain of ' gcb ' exceeds the fixed-point range.']);
      |         end
      |         if f32PropGain<-2^31
      |           f32PropGain=-2^31;
      |           warning(['Parameter f32PropGain of ' gcb ' exceeds the fixed-point range.']);
      |         end
      |         s16IntegGainShift=ceil(log2(abs(kif)));
      |         if s16IntegGainShift<-31
      |           s16IntegGainShift=-31;
      |         end
      |         if s16IntegGainShift>31
      |           s16IntegGainShift=31;
      |           warning(['Parameter s16IntegGainShift of ' gcb ' exceeds the fixed-point range.']);
      |         end
      |         f32IntegGain=round(kif*2^(-s16IntegGainShift)*2^31);
      |         if f32IntegGain>2^31-1
      |           f32IntegGain=2^31-1;
      |           warning(['Parameter f32IntegGain of ' gcb ' exceeds the fixed-point range.']);
      |         end
      |         if f32IntegGain<-2^31
      |           f32IntegGain=-2^31;
      |           warning(['Parameter f32IntegGain of ' gcb ' exceeds the fixed-point range.']);
      |         end
      |         if (Idmax<0)
      |           iratio=abs(Idmax)/iscale;
      |           lowlim=0.3183098861837907*acos(iratio)-0.5;
      |         else
      |           lowlim=0.0;
      |         end
      |         f32LowerLimit=round(lowlim*2^31);
      |         if f32LowerLimit>2^31-1
      |           f32LowerLimit=2^31-1;
      |           warning(['Parameter f32LowerLimit of ' gcb ' exceeds the fixed-point range.']);
      |         end
      |         if f32LowerLimit<-2^31
      |           f32LowerLimit=-2^31;
      |           warning(['Parameter f32LowerLimit of ' gcb ' exceeds the fixed-point range.']);
      |         end
      |         f32UpperLimit=0;
      |         u16NSamples=round(log2(1.0/abs(lambdaFW)));
      |         if u16NSamples>31
      |           u16NSamples=31;
      |         end
      |         if u16NSamples<0
      |           u16NSamples=0;
      |         end
      |         if isnan(u16NSamples)
      |           if ~strcmp(u16NSamples_bkup,'0')
      |             set_param(gcb,'u16NSamples','0');
      |           end
      |         else
      |           tmps=num2str(u16NSamples);
      |           if ~strcmp(u16NSamples_bkup,tmps)
      |             set_param(gcb,'u16NSamples',tmps);
      |           end
      |         end
      |         if isnan(f32PropGain)
      |           if ~strcmp(f32PropGain_bkup,'0')
      |             set_param(gcb,'f32PropGain','0');
      |           end
      |         else
      |           tmps=num2str(f32PropGain);
      |           if ~strcmp(f32PropGain_bkup,tmps)
      |             set_param(gcb,'f32PropGain',tmps);
      |           end
      |         end
      |         if isnan(f32IntegGain)
      |           if ~strcmp(f32IntegGain_bkup,'0')
      |             set_param(gcb,'f32IntegGain','0');
      |           end
      |         else
      |           tmps=num2str(f32IntegGain);
      |           if ~strcmp(f32IntegGain_bkup,tmps)
      |             set_param(gcb,'f32IntegGain',tmps);
      |           end
      |         end
      |         if isnan(s16PropGainShift)
      |           if ~strcmp(s16PropGainShift_bkup,'0')
      |             set_param(gcb,'s16PropGainShift','0');
      |           end
      |         else
      |           tmps=num2str(s16PropGainShift);
      |           if ~strcmp(s16PropGainShift_bkup,tmps)
      |             set_param(gcb,'s16PropGainShift',tmps);
      |           end
      |         end
      |         if isnan(s16IntegGainShift)
      |           if ~strcmp(s16IntegGainShift_bkup,'0')
      |             set_param(gcb,'s16IntegGainShift','0');
      |           end
      |         else
      |           tmps=num2str(s16IntegGainShift);
      |           if ~strcmp(s16IntegGainShift_bkup,tmps)
      |             set_param(gcb,'s16IntegGainShift',tmps);
      |           end
      |         end
      |         if isnan(f32LowerLimit)
      |           if ~strcmp(f32LowerLimit_bkup,'0')
      |             set_param(gcb,'f32LowerLimit','0');
      |           end
      |         else
      |           tmps=num2str(f32LowerLimit);
      |           if ~strcmp(f32LowerLimit_bkup,tmps)
      |             set_param(gcb,'f32LowerLimit',tmps);
      |           end
      |         end
      |         if isnan(f32UpperLimit)
      |           if ~strcmp(f32UpperLimit_bkup,'0')
      |             set_param(gcb,'f32UpperLimit','0');
      |           end
      |         else
      |           tmps=num2str(f32UpperLimit);
      |           if ~strcmp(f32UpperLimit_bkup,tmps)
      |             set_param(gcb,'f32UpperLimit',tmps);
      |           end
      |         end
      |       end
      |     end
      |   catch
      |    warning(['Sample time cannot be calculated for the block ' gcb])
      |   end
      | end
      mask DialogControl timeHint Prompt: Note: Implementation parameters cannot be calculated yet because the block's inherited sample time is unknown. Simulink will update the sample time when you run the simulation.
      mask Display:
      | color('black');
      | pos = get_param(gcb, 'Position');
      | width = pos(3) - pos(1);
      | height = pos(4) - pos(2);
      | tX=width/2;
      | tY=height - 25;
      | color('black');
      | text(tX,tY, 'AMCLIB_FW_F32', 'horizontalAlignment', 'center');
      | if showStates == 2
      |   color('red');
      |   text(tX,tY - 20, ['debugging mode' char(13) char(10) '(limited performance)'], 'horizontalAlignment', 'center');
      | end
  AMCLIB_FluxEstimAB_F32 : Subsystem  TreatAsAtomicUnit=on  mask(AMCLIB_FluxEstimAB_F32){showStates=Hide (faster execution), Rs=0.33, Ls=6e-4, mechspeed=3000, polepairs=1, uscale=15, iscale=10, autoCalcEn=on, f32KRs=0, f32KLs=0, u16NShift=0}
      mask prompts: showStates "Show parameters as inputs:"; Rs "Winding resistance Rs [ohm]:"; Ls "Stator inductance Ls [H]"; mechspeed "Maximum mechanical speed of the motor [RPM]:"; polepairs "Number of pole pairs of the motor:"; uscale "U_max (maximum DC bus voltage) [V]:"; iscale "I_max (maximum phase current) [A]:"; autoCalcEn "Calculate implementation parameters from physical parameters"; f32KRs "f32KRs (Scaled stator resistance):"; f32KLs "f32KLs (Scaled stator inductance):"; u16NShift "u16NShift (Scaling bitwise shift applied to the coefficients):"
      mask help: This block calculates the PMSM rotor position by estimating the rotor flux in the Alpha-Beta reference frame. The function can be used for sensorless FOC in 32-bit fixed-point fractional implementation.
      mask init:
      | ddName = get_param(bdroot,'DataDictionary');
      | if length(ddName)==0
      |   set_param(bdroot,'DataDictionary','ammclib_types.sldd');
      | else
      |   dd = Simulink.data.dictionary.open(ddName);
      |   data = getSection(dd,'Design Data');
      |   if ~exist(data,'SWLIBS_2Syst_F16')
      |     addDataSource(dd,'ammclib_types.sldd');
      |     saveChanges(dd);
      |   end
      | end
      | 
      | if showStates == 1
      |   % hidden state variables
      |   if strcmp(get_param([gcb '/f32KRs'], 'BlockType'), 'Inport')
      |     posblk = get_param(gcb, 'Position');
      | 
      |     pos = get_param([gcb, '/f32KRs'], 'Position');
      |     orient = get_param([gcb, '/f32KRs'], 'Orientation');
      |     delete_block([gcb, '/f32KRs']);
      |     add_block('built-in/Ground', [gcb, '/f32KRs'], 'Position', pos, 'Orientation', orient);
      | 
      |     pos = get_param([gcb, '/f32KLs'], 'Position');
      |     orient = get_param([gcb, '/f32KLs'], 'Orientation');
      |     delete_block([gcb, '/f32KLs']);
      |     add_block('built-in/Ground', [gcb, '/f32KLs'], 'Position', pos, 'Orientation', orient);
      | 
      |     pos = get_param([gcb, '/u16NShift'], 'Position');
      |     orient = get_param([gcb, '/u16NShift'], 'Orientation');
      |     delete_block([gcb, '/u16NShift']);
      |     add_block('built-in/Ground', [gcb, '/u16NShift'], 'Position', pos, 'Orientation', orient);
      | 
      | 
      | 
      |     set_param([gcb '/f32Velocity'], 'Port', '1');
      |     set_param([gcb '/pIAB'], 'Port', '2');
      |     set_param([gcb '/pUAB'], 'Port', '3');
      | 
      |     tmpOutCnt=0;
      |     tmpOutCnt=tmpOutCnt+1;
      |     set_param([gcb '/f32Phase'], 'Port', num2str(tmpOutCnt));
      | 
      |     autoCalcEn=get_param(gcb,'autoCalcEn');
      |     if strcmp(autoCalcEn,'on')
      |       set_param(gcb,'MaskEnables',{'on','on','on','on','on','on','on','on','on','on','on'});
      |     else
      |       set_param(gcb,'MaskEnables',{'on','off','off','off','off','off','off','on','on','on','on'});
      |     end
      | 
      |     if (posblk(4) - posblk(2)) > 100
      |       height = 100;
      |       set_param(gcb,'Position',[posblk(1), posblk(2), posblk(3), posblk(2)+height])
      |     end
      |   end
      | else
      |   % shown state variables
      |   if strcmp(get_param([gcb '/f32KRs'], 'BlockType'), 'Ground')
      |     posblk = get_param(gcb, 'Position');
      | 
      |     pos = get_param([gcb, '/f32KRs'], 'Position');
      |     orient = get_param([gcb, '/f32KRs'], 'Orientation');
      |     delete_block([gcb, '/f32KRs']);
      |     add_block('built-in/Inport', [gcb, '/f32KRs'], 'Position', pos, 'Orientation', orient, 'OutDataTypeStr', 'int32');
      | 
      |     pos = get_param([gcb, '/f32KLs'], 'Position');
      |     orient = get_param([gcb, '/f32KLs'], 'Orientation');
      |     delete_block([gcb, '/f32KLs']);
      |     add_block('built-in/Inport', [gcb, '/f32KLs'], 'Position', pos, 'Orientation', orient, 'OutDataTypeStr', 'int32');
      | 
      |     pos = get_param([gcb, '/u16NShift'], 'Position');
      |     orient = get_param([gcb, '/u16NShift'], 'Orientation');
      |     delete_block([gcb, '/u16NShift']);
      |     add_block('built-in/Inport', [gcb, '/u16NShift'], 'Position', pos, 'Orientation', orient, 'OutDataTypeStr', 'uint16');
      | 
      | 
      | 
      | 
      | 
      |     set_param([gcb '/f32Velocity'], 'Port', '1');
      |     set_param([gcb '/pIAB'], 'Port', '2');
      |     set_param([gcb '/pUAB'], 'Port', '3');
      |     set_param([gcb '/f32KRs'], 'Port', '4');
      |     set_param([gcb '/f32KLs'], 'Port', '5');
      |     set_param([gcb '/u16NShift'], 'Port', '6');
      | 
      |     tmpOutCnt=0;
      |     tmpOutCnt=tmpOutCnt+1;
      |     set_param([gcb '/f32Phase'], 'Port', num2str(tmpOutCnt));
      | 
      |     set_param(gcb,'MaskEnables',{'on','off','off','off','off','off','off','off','off','off','off'});
      | 
      |     if (posblk(4) - posblk(2)) < 175
      |       height = 175;
      |       set_param(gcb,'Position',[posblk(1), posblk(2), posblk(3), posblk(2)+height])
      |     end
      |   end
      | end
      settings: RTWSystemCode=Inline
      mask Help: web([fileparts(which('ammclib_bam_S32K3xx.slx')) '/../doc/S32K3XXMCLUG.pdf'], '-browser')
      mask TypeOptions showStates: Hide (faster execution) | Show (parameters can be changed during simulation)
      mask Callback showStates:
      | maskStr=get_param(gcb,'showStates');
      | if strcmp(maskStr,'Hide (faster execution)')
      |   if strcmp(get_param([gcb '/f32KRs'], 'BlockType'), 'Inport')
      |     autoCalcEn=get_param(gcb,'autoCalcEn');
      |     if strcmp(autoCalcEn,'on')
      |       set_param(gcb,'MaskEnables',{'on','on','on','on','on','on','on','on','on','on','on'});
      |     else
      |       set_param(gcb,'MaskEnables',{'on','off','off','off','off','off','off','on','on','on','on'});
      |     end
      |   end
      | else
      |   if strcmp(get_param([gcb '/f32KRs'], 'BlockType'), 'Ground')
      |     set_param(gcb,'MaskEnables',{'on','off','off','off','off','off','off','off','off','off','off'});
      |   end
      | end
      mask Callback Rs:
      | autoCalcEn=get_param(gcb,'autoCalcEn');
      | if strcmp(autoCalcEn,'on')
      |   f32KRs_bkup=get_param(gcb,'f32KRs');
      |   f32KLs_bkup=get_param(gcb,'f32KLs');
      |   u16NShift_bkup=get_param(gcb,'u16NShift');
      |   Rs=Simulink.data.evalinGlobal(bdroot,get_param(gcb,'Rs'));
      |   Ls=Simulink.data.evalinGlobal(bdroot,get_param(gcb,'Ls'));
      |   mechspeed=Simulink.data.evalinGlobal(bdroot,get_param(gcb,'mechspeed'));
      |   polepairs=Simulink.data.evalinGlobal(bdroot,get_param(gcb,'polepairs'));
      |   uscale=Simulink.data.evalinGlobal(bdroot,get_param(gcb,'uscale'));
      |   iscale=Simulink.data.evalinGlobal(bdroot,get_param(gcb,'iscale'));
      |   if (Ls<=0)
      |     warning('Inductance Ls must be positive.');
      |   end
      |   if (Rs<0)
      |     warning('Resistance Rs must be non-negative.');
      |   end
      |   if (mechspeed<=0)
      |     warning('Max. speed must be positive.');
      |   end
      |   if (polepairs<1)
      |     warning('Number of pole pairs must be a natural number (1, 2, 3, ...).');
      |   end
      |   if (round(polepairs)~=polepairs)
      |     warning('Number of pole pairs must be a natural number (1, 2, 3, ...).');
      |   end
      |   if (uscale<=0)
      |     warning('U_max must be positive.');
      |   end
      |   if (iscale<=0)
      |     warning('I_max must be positive.');
      |   end
      |   wmax=polepairs*mechspeed*1.047197551196598e-01;
      |   Rssc=Rs*iscale/uscale;
      |   Lssc=Ls*wmax*iscale/uscale;
      |   u16NShift=ceil(log2(abs(Rssc)));
      |   tmpsh=ceil(log2(abs(Lssc)));
      |   if u16NShift<tmpsh
      |     u16NShift=tmpsh;
      |   end
      |   if u16NShift<0
      |     u16NShift=0;
      |   end
      |   if u16NShift>31
      |     u16NShift=31;
      |     warning(['Parameter u16NShift of ' gcb ' exceeds the fixed-point range.']);
      |   end
      |   f32KRs=round(Rssc*2^(-u16NShift)*2^31);
      |   if f32KRs>2^31-1
      |     f32KRs=2^31-1;
      |     warning(['Parameter f32KRs of ' gcb ' exceeds the fixed-point range.']);
      |   end
      |   if f32KRs<-2^31
      |     f32KRs=-2^31;
      |     warning(['Parameter f32KRs of ' gcb ' exceeds the fixed-point range.']);
      |   end
      |   f32KLs=round(Lssc*2^(-u16NShift)*2^31);
      |   if f32KLs>2^31-1
      |     f32KLs=2^31-1;
      |     warning(['Parameter f32KLs of ' gcb ' exceeds the fixed-point range.']);
      |   end
      |   if f32KLs<-2^31
      |     f32KLs=-2^31;
      |     warning(['Parameter f32KLs of ' gcb ' exceeds the fixed-point range.']);
      |   end
      |   if isnan(f32KRs)
      |     if ~strcmp(f32KRs_bkup,'0')
      |       set_param(gcb,'f32KRs','0');
      |     end
      |   else
      |     tmps=num2str(f32KRs);
      |     if ~strcmp(f32KRs_bkup,tmps)
      |       set_param(gcb,'f32KRs',tmps);
      |     end
      |   end
      |   if isnan(f32KLs)
      |     if ~strcmp(f32KLs_bkup,'0')
      |       set_param(gcb,'f32KLs','0');
      |     end
      |   else
      |     tmps=num2str(f32KLs);
      |     if ~strcmp(f32KLs_bkup,tmps)
      |       set_param(gcb,'f32KLs',tmps);
      |     end
      |   end
      |   if isnan(u16NShift)
      |     if ~strcmp(u16NShift_bkup,'0')
      |       set_param(gcb,'u16NShift','0');
      |     end
      |   else
      |     tmps=num2str(u16NShift);
      |     if ~strcmp(u16NShift_bkup,tmps)
      |       set_param(gcb,'u16NShift',tmps);
      |     end
      |   end
      | end
      mask Callback Ls:
      | autoCalcEn=get_param(gcb,'autoCalcEn');
      | if strcmp(autoCalcEn,'on')
      |   f32KRs_bkup=get_param(gcb,'f32KRs');
      |   f32KLs_bkup=get_param(gcb,'f32KLs');
      |   u16NShift_bkup=get_param(gcb,'u16NShift');
      |   Rs=Simulink.data.evalinGlobal(bdroot,get_param(gcb,'Rs'));
      |   Ls=Simulink.data.evalinGlobal(bdroot,get_param(gcb,'Ls'));
      |   mechspeed=Simulink.data.evalinGlobal(bdroot,get_param(gcb,'mechspeed'));
      |   polepairs=Simulink.data.evalinGlobal(bdroot,get_param(gcb,'polepairs'));
      |   uscale=Simulink.data.evalinGlobal(bdroot,get_param(gcb,'uscale'));
      |   iscale=Simulink.data.evalinGlobal(bdroot,get_param(gcb,'iscale'));
      |   if (Ls<=0)
      |     warning('Inductance Ls must be positive.');
      |   end
      |   if (Rs<0)
      |     warning('Resistance Rs must be non-negative.');
      |   end
      |   if (mechspeed<=0)
      |     warning('Max. speed must be positive.');
      |   end
      |   if (polepairs<1)
      |     warning('Number of pole pairs must be a natural number (1, 2, 3, ...).');
      |   end
      |   if (round(polepairs)~=polepairs)
      |     warning('Number of pole pairs must be a natural number (1, 2, 3, ...).');
      |   end
      |   if (uscale<=0)
      |     warning('U_max must be positive.');
      |   end
      |   if (iscale<=0)
      |     warning('I_max must be positive.');
      |   end
      |   wmax=polepairs*mechspeed*1.047197551196598e-01;
      |   Rssc=Rs*iscale/uscale;
      |   Lssc=Ls*wmax*iscale/uscale;
      |   u16NShift=ceil(log2(abs(Rssc)));
      |   tmpsh=ceil(log2(abs(Lssc)));
      |   if u16NShift<tmpsh
      |     u16NShift=tmpsh;
      |   end
      |   if u16NShift<0
      |     u16NShift=0;
      |   end
      |   if u16NShift>31
      |     u16NShift=31;
      |     warning(['Parameter u16NShift of ' gcb ' exceeds the fixed-point range.']);
      |   end
      |   f32KRs=round(Rssc*2^(-u16NShift)*2^31);
      |   if f32KRs>2^31-1
      |     f32KRs=2^31-1;
      |     warning(['Parameter f32KRs of ' gcb ' exceeds the fixed-point range.']);
      |   end
      |   if f32KRs<-2^31
      |     f32KRs=-2^31;
      |     warning(['Parameter f32KRs of ' gcb ' exceeds the fixed-point range.']);
      |   end
      |   f32KLs=round(Lssc*2^(-u16NShift)*2^31);
      |   if f32KLs>2^31-1
      |     f32KLs=2^31-1;
      |     warning(['Parameter f32KLs of ' gcb ' exceeds the fixed-point range.']);
      |   end
      |   if f32KLs<-2^31
      |     f32KLs=-2^31;
      |     warning(['Parameter f32KLs of ' gcb ' exceeds the fixed-point range.']);
      |   end
      |   if isnan(f32KRs)
      |     if ~strcmp(f32KRs_bkup,'0')
      |       set_param(gcb,'f32KRs','0');
      |     end
      |   else
      |     tmps=num2str(f32KRs);
      |     if ~strcmp(f32KRs_bkup,tmps)
      |       set_param(gcb,'f32KRs',tmps);
      |     end
      |   end
      |   if isnan(f32KLs)
      |     if ~strcmp(f32KLs_bkup,'0')
      |       set_param(gcb,'f32KLs','0');
      |     end
      |   else
      |     tmps=num2str(f32KLs);
      |     if ~strcmp(f32KLs_bkup,tmps)
      |       set_param(gcb,'f32KLs',tmps);
      |     end
      |   end
      |   if isnan(u16NShift)
      |     if ~strcmp(u16NShift_bkup,'0')
      |       set_param(gcb,'u16NShift','0');
      |     end
      |   else
      |     tmps=num2str(u16NShift);
      |     if ~strcmp(u16NShift_bkup,tmps)
      |       set_param(gcb,'u16NShift',tmps);
      |     end
      |   end
      | end
      mask Callback mechspeed:
      | autoCalcEn=get_param(gcb,'autoCalcEn');
      | if strcmp(autoCalcEn,'on')
      |   f32KRs_bkup=get_param(gcb,'f32KRs');
      |   f32KLs_bkup=get_param(gcb,'f32KLs');
      |   u16NShift_bkup=get_param(gcb,'u16NShift');
      |   Rs=Simulink.data.evalinGlobal(bdroot,get_param(gcb,'Rs'));
      |   Ls=Simulink.data.evalinGlobal(bdroot,get_param(gcb,'Ls'));
      |   mechspeed=Simulink.data.evalinGlobal(bdroot,get_param(gcb,'mechspeed'));
      |   polepairs=Simulink.data.evalinGlobal(bdroot,get_param(gcb,'polepairs'));
      |   uscale=Simulink.data.evalinGlobal(bdroot,get_param(gcb,'uscale'));
      |   iscale=Simulink.data.evalinGlobal(bdroot,get_param(gcb,'iscale'));
      |   if (Ls<=0)
      |     warning('Inductance Ls must be positive.');
      |   end
      |   if (Rs<0)
      |     warning('Resistance Rs must be non-negative.');
      |   end
      |   if (mechspeed<=0)
      |     warning('Max. speed must be positive.');
      |   end
      |   if (polepairs<1)
      |     warning('Number of pole pairs must be a natural number (1, 2, 3, ...).');
      |   end
      |   if (round(polepairs)~=polepairs)
      |     warning('Number of pole pairs must be a natural number (1, 2, 3, ...).');
      |   end
      |   if (uscale<=0)
      |     warning('U_max must be positive.');
      |   end
      |   if (iscale<=0)
      |     warning('I_max must be positive.');
      |   end
      |   wmax=polepairs*mechspeed*1.047197551196598e-01;
      |   Rssc=Rs*iscale/uscale;
      |   Lssc=Ls*wmax*iscale/uscale;
      |   u16NShift=ceil(log2(abs(Rssc)));
      |   tmpsh=ceil(log2(abs(Lssc)));
      |   if u16NShift<tmpsh
      |     u16NShift=tmpsh;
      |   end
      |   if u16NShift<0
      |     u16NShift=0;
      |   end
      |   if u16NShift>31
      |     u16NShift=31;
      |     warning(['Parameter u16NShift of ' gcb ' exceeds the fixed-point range.']);
      |   end
      |   f32KRs=round(Rssc*2^(-u16NShift)*2^31);
      |   if f32KRs>2^31-1
      |     f32KRs=2^31-1;
      |     warning(['Parameter f32KRs of ' gcb ' exceeds the fixed-point range.']);
      |   end
      |   if f32KRs<-2^31
      |     f32KRs=-2^31;
      |     warning(['Parameter f32KRs of ' gcb ' exceeds the fixed-point range.']);
      |   end
      |   f32KLs=round(Lssc*2^(-u16NShift)*2^31);
      |   if f32KLs>2^31-1
      |     f32KLs=2^31-1;
      |     warning(['Parameter f32KLs of ' gcb ' exceeds the fixed-point range.']);
      |   end
      |   if f32KLs<-2^31
      |     f32KLs=-2^31;
      |     warning(['Parameter f32KLs of ' gcb ' exceeds the fixed-point range.']);
      |   end
      |   if isnan(f32KRs)
      |     if ~strcmp(f32KRs_bkup,'0')
      |       set_param(gcb,'f32KRs','0');
      |     end
      |   else
      |     tmps=num2str(f32KRs);
      |     if ~strcmp(f32KRs_bkup,tmps)
      |       set_param(gcb,'f32KRs',tmps);
      |     end
      |   end
      |   if isnan(f32KLs)
      |     if ~strcmp(f32KLs_bkup,'0')
      |       set_param(gcb,'f32KLs','0');
      |     end
      |   else
      |     tmps=num2str(f32KLs);
      |     if ~strcmp(f32KLs_bkup,tmps)
      |       set_param(gcb,'f32KLs',tmps);
      |     end
      |   end
      |   if isnan(u16NShift)
      |     if ~strcmp(u16NShift_bkup,'0')
      |       set_param(gcb,'u16NShift','0');
      |     end
      |   else
      |     tmps=num2str(u16NShift);
      |     if ~strcmp(u16NShift_bkup,tmps)
      |       set_param(gcb,'u16NShift',tmps);
      |     end
      |   end
      | end
      mask Callback polepairs:
      | autoCalcEn=get_param(gcb,'autoCalcEn');
      | if strcmp(autoCalcEn,'on')
      |   f32KRs_bkup=get_param(gcb,'f32KRs');
      |   f32KLs_bkup=get_param(gcb,'f32KLs');
      |   u16NShift_bkup=get_param(gcb,'u16NShift');
      |   Rs=Simulink.data.evalinGlobal(bdroot,get_param(gcb,'Rs'));
      |   Ls=Simulink.data.evalinGlobal(bdroot,get_param(gcb,'Ls'));
      |   mechspeed=Simulink.data.evalinGlobal(bdroot,get_param(gcb,'mechspeed'));
      |   polepairs=Simulink.data.evalinGlobal(bdroot,get_param(gcb,'polepairs'));
      |   uscale=Simulink.data.evalinGlobal(bdroot,get_param(gcb,'uscale'));
      |   iscale=Simulink.data.evalinGlobal(bdroot,get_param(gcb,'iscale'));
      |   if (Ls<=0)
      |     warning('Inductance Ls must be positive.');
      |   end
      |   if (Rs<0)
      |     warning('Resistance Rs must be non-negative.');
      |   end
      |   if (mechspeed<=0)
      |     warning('Max. speed must be positive.');
      |   end
      |   if (polepairs<1)
      |     warning('Number of pole pairs must be a natural number (1, 2, 3, ...).');
      |   end
      |   if (round(polepairs)~=polepairs)
      |     warning('Number of pole pairs must be a natural number (1, 2, 3, ...).');
      |   end
      |   if (uscale<=0)
      |     warning('U_max must be positive.');
      |   end
      |   if (iscale<=0)
      |     warning('I_max must be positive.');
      |   end
      |   wmax=polepairs*mechspeed*1.047197551196598e-01;
      |   Rssc=Rs*iscale/uscale;
      |   Lssc=Ls*wmax*iscale/uscale;
      |   u16NShift=ceil(log2(abs(Rssc)));
      |   tmpsh=ceil(log2(abs(Lssc)));
      |   if u16NShift<tmpsh
      |     u16NShift=tmpsh;
      |   end
      |   if u16NShift<0
      |     u16NShift=0;
      |   end
      |   if u16NShift>31
      |     u16NShift=31;
      |     warning(['Parameter u16NShift of ' gcb ' exceeds the fixed-point range.']);
      |   end
      |   f32KRs=round(Rssc*2^(-u16NShift)*2^31);
      |   if f32KRs>2^31-1
      |     f32KRs=2^31-1;
      |     warning(['Parameter f32KRs of ' gcb ' exceeds the fixed-point range.']);
      |   end
      |   if f32KRs<-2^31
      |     f32KRs=-2^31;
      |     warning(['Parameter f32KRs of ' gcb ' exceeds the fixed-point range.']);
      |   end
      |   f32KLs=round(Lssc*2^(-u16NShift)*2^31);
      |   if f32KLs>2^31-1
      |     f32KLs=2^31-1;
      |     warning(['Parameter f32KLs of ' gcb ' exceeds the fixed-point range.']);
      |   end
      |   if f32KLs<-2^31
      |     f32KLs=-2^31;
      |     warning(['Parameter f32KLs of ' gcb ' exceeds the fixed-point range.']);
      |   end
      |   if isnan(f32KRs)
      |     if ~strcmp(f32KRs_bkup,'0')
      |       set_param(gcb,'f32KRs','0');
      |     end
      |   else
      |     tmps=num2str(f32KRs);
      |     if ~strcmp(f32KRs_bkup,tmps)
      |       set_param(gcb,'f32KRs',tmps);
      |     end
      |   end
      |   if isnan(f32KLs)
      |     if ~strcmp(f32KLs_bkup,'0')
      |       set_param(gcb,'f32KLs','0');
      |     end
      |   else
      |     tmps=num2str(f32KLs);
      |     if ~strcmp(f32KLs_bkup,tmps)
      |       set_param(gcb,'f32KLs',tmps);
      |     end
      |   end
      |   if isnan(u16NShift)
      |     if ~strcmp(u16NShift_bkup,'0')
      |       set_param(gcb,'u16NShift','0');
      |     end
      |   else
      |     tmps=num2str(u16NShift);
      |     if ~strcmp(u16NShift_bkup,tmps)
      |       set_param(gcb,'u16NShift',tmps);
      |     end
      |   end
      | end
      mask Callback uscale:
      | autoCalcEn=get_param(gcb,'autoCalcEn');
      | if strcmp(autoCalcEn,'on')
      |   f32KRs_bkup=get_param(gcb,'f32KRs');
      |   f32KLs_bkup=get_param(gcb,'f32KLs');
      |   u16NShift_bkup=get_param(gcb,'u16NShift');
      |   Rs=Simulink.data.evalinGlobal(bdroot,get_param(gcb,'Rs'));
      |   Ls=Simulink.data.evalinGlobal(bdroot,get_param(gcb,'Ls'));
      |   mechspeed=Simulink.data.evalinGlobal(bdroot,get_param(gcb,'mechspeed'));
      |   polepairs=Simulink.data.evalinGlobal(bdroot,get_param(gcb,'polepairs'));
      |   uscale=Simulink.data.evalinGlobal(bdroot,get_param(gcb,'uscale'));
      |   iscale=Simulink.data.evalinGlobal(bdroot,get_param(gcb,'iscale'));
      |   if (Ls<=0)
      |     warning('Inductance Ls must be positive.');
      |   end
      |   if (Rs<0)
      |     warning('Resistance Rs must be non-negative.');
      |   end
      |   if (mechspeed<=0)
      |     warning('Max. speed must be positive.');
      |   end
      |   if (polepairs<1)
      |     warning('Number of pole pairs must be a natural number (1, 2, 3, ...).');
      |   end
      |   if (round(polepairs)~=polepairs)
      |     warning('Number of pole pairs must be a natural number (1, 2, 3, ...).');
      |   end
      |   if (uscale<=0)
      |     warning('U_max must be positive.');
      |   end
      |   if (iscale<=0)
      |     warning('I_max must be positive.');
      |   end
      |   wmax=polepairs*mechspeed*1.047197551196598e-01;
      |   Rssc=Rs*iscale/uscale;
      |   Lssc=Ls*wmax*iscale/uscale;
      |   u16NShift=ceil(log2(abs(Rssc)));
      |   tmpsh=ceil(log2(abs(Lssc)));
      |   if u16NShift<tmpsh
      |     u16NShift=tmpsh;
      |   end
      |   if u16NShift<0
      |     u16NShift=0;
      |   end
      |   if u16NShift>31
      |     u16NShift=31;
      |     warning(['Parameter u16NShift of ' gcb ' exceeds the fixed-point range.']);
      |   end
      |   f32KRs=round(Rssc*2^(-u16NShift)*2^31);
      |   if f32KRs>2^31-1
      |     f32KRs=2^31-1;
      |     warning(['Parameter f32KRs of ' gcb ' exceeds the fixed-point range.']);
      |   end
      |   if f32KRs<-2^31
      |     f32KRs=-2^31;
      |     warning(['Parameter f32KRs of ' gcb ' exceeds the fixed-point range.']);
      |   end
      |   f32KLs=round(Lssc*2^(-u16NShift)*2^31);
      |   if f32KLs>2^31-1
      |     f32KLs=2^31-1;
      |     warning(['Parameter f32KLs of ' gcb ' exceeds the fixed-point range.']);
      |   end
      |   if f32KLs<-2^31
      |     f32KLs=-2^31;
      |     warning(['Parameter f32KLs of ' gcb ' exceeds the fixed-point range.']);
      |   end
      |   if isnan(f32KRs)
      |     if ~strcmp(f32KRs_bkup,'0')
      |       set_param(gcb,'f32KRs','0');
      |     end
      |   else
      |     tmps=num2str(f32KRs);
      |     if ~strcmp(f32KRs_bkup,tmps)
      |       set_param(gcb,'f32KRs',tmps);
      |     end
      |   end
      |   if isnan(f32KLs)
      |     if ~strcmp(f32KLs_bkup,'0')
      |       set_param(gcb,'f32KLs','0');
      |     end
      |   else
      |     tmps=num2str(f32KLs);
      |     if ~strcmp(f32KLs_bkup,tmps)
      |       set_param(gcb,'f32KLs',tmps);
      |     end
      |   end
      |   if isnan(u16NShift)
      |     if ~strcmp(u16NShift_bkup,'0')
      |       set_param(gcb,'u16NShift','0');
      |     end
      |   else
      |     tmps=num2str(u16NShift);
      |     if ~strcmp(u16NShift_bkup,tmps)
      |       set_param(gcb,'u16NShift',tmps);
      |     end
      |   end
      | end
      mask Callback iscale:
      | autoCalcEn=get_param(gcb,'autoCalcEn');
      | if strcmp(autoCalcEn,'on')
      |   f32KRs_bkup=get_param(gcb,'f32KRs');
      |   f32KLs_bkup=get_param(gcb,'f32KLs');
      |   u16NShift_bkup=get_param(gcb,'u16NShift');
      |   Rs=Simulink.data.evalinGlobal(bdroot,get_param(gcb,'Rs'));
      |   Ls=Simulink.data.evalinGlobal(bdroot,get_param(gcb,'Ls'));
      |   mechspeed=Simulink.data.evalinGlobal(bdroot,get_param(gcb,'mechspeed'));
      |   polepairs=Simulink.data.evalinGlobal(bdroot,get_param(gcb,'polepairs'));
      |   uscale=Simulink.data.evalinGlobal(bdroot,get_param(gcb,'uscale'));
      |   iscale=Simulink.data.evalinGlobal(bdroot,get_param(gcb,'iscale'));
      |   if (Ls<=0)
      |     warning('Inductance Ls must be positive.');
      |   end
      |   if (Rs<0)
      |     warning('Resistance Rs must be non-negative.');
      |   end
      |   if (mechspeed<=0)
      |     warning('Max. speed must be positive.');
      |   end
      |   if (polepairs<1)
      |     warning('Number of pole pairs must be a natural number (1, 2, 3, ...).');
      |   end
      |   if (round(polepairs)~=polepairs)
      |     warning('Number of pole pairs must be a natural number (1, 2, 3, ...).');
      |   end
      |   if (uscale<=0)
      |     warning('U_max must be positive.');
      |   end
      |   if (iscale<=0)
      |     warning('I_max must be positive.');
      |   end
      |   wmax=polepairs*mechspeed*1.047197551196598e-01;
      |   Rssc=Rs*iscale/uscale;
      |   Lssc=Ls*wmax*iscale/uscale;
      |   u16NShift=ceil(log2(abs(Rssc)));
      |   tmpsh=ceil(log2(abs(Lssc)));
      |   if u16NShift<tmpsh
      |     u16NShift=tmpsh;
      |   end
      |   if u16NShift<0
      |     u16NShift=0;
      |   end
      |   if u16NShift>31
      |     u16NShift=31;
      |     warning(['Parameter u16NShift of ' gcb ' exceeds the fixed-point range.']);
      |   end
      |   f32KRs=round(Rssc*2^(-u16NShift)*2^31);
      |   if f32KRs>2^31-1
      |     f32KRs=2^31-1;
      |     warning(['Parameter f32KRs of ' gcb ' exceeds the fixed-point range.']);
      |   end
      |   if f32KRs<-2^31
      |     f32KRs=-2^31;
      |     warning(['Parameter f32KRs of ' gcb ' exceeds the fixed-point range.']);
      |   end
      |   f32KLs=round(Lssc*2^(-u16NShift)*2^31);
      |   if f32KLs>2^31-1
      |     f32KLs=2^31-1;
      |     warning(['Parameter f32KLs of ' gcb ' exceeds the fixed-point range.']);
      |   end
      |   if f32KLs<-2^31
      |     f32KLs=-2^31;
      |     warning(['Parameter f32KLs of ' gcb ' exceeds the fixed-point range.']);
      |   end
      |   if isnan(f32KRs)
      |     if ~strcmp(f32KRs_bkup,'0')
      |       set_param(gcb,'f32KRs','0');
      |     end
      |   else
      |     tmps=num2str(f32KRs);
      |     if ~strcmp(f32KRs_bkup,tmps)
      |       set_param(gcb,'f32KRs',tmps);
      |     end
      |   end
      |   if isnan(f32KLs)
      |     if ~strcmp(f32KLs_bkup,'0')
      |       set_param(gcb,'f32KLs','0');
      |     end
      |   else
      |     tmps=num2str(f32KLs);
      |     if ~strcmp(f32KLs_bkup,tmps)
      |       set_param(gcb,'f32KLs',tmps);
      |     end
      |   end
      |   if isnan(u16NShift)
      |     if ~strcmp(u16NShift_bkup,'0')
      |       set_param(gcb,'u16NShift','0');
      |     end
      |   else
      |     tmps=num2str(u16NShift);
      |     if ~strcmp(u16NShift_bkup,tmps)
      |       set_param(gcb,'u16NShift',tmps);
      |     end
      |   end
      | end
      mask Callback autoCalcEn:
      | maskStr=get_param(gcb,'showStates');
      | if strcmp(maskStr,'Hide (faster execution)')
      |   p=Simulink.Mask.get(gcb);
      |   autoCalcEn=get_param(gcb,'autoCalcEn');
      |   hintText=p.getDialogControl('timeHint');
      |   if strcmp(autoCalcEn,'on')
      |     param=p.getParameter('iscale');
      |     if strcmp(param.Enabled,'off')
      |       p=Simulink.Mask.get(gcb);
      |       param=p.getParameter('Rs');
      |       param.set('Enabled','on');
      |       param=p.getParameter('Ls');
      |       param.set('Enabled','on');
      |       param=p.getParameter('mechspeed');
      |       param.set('Enabled','on');
      |       param=p.getParameter('polepairs');
      |       param.set('Enabled','on');
      |       param=p.getParameter('uscale');
      |       param.set('Enabled','on');
      |       param=p.getParameter('iscale');
      |       param.set('Enabled','on');
      |     end
      |     f32KRs_bkup=get_param(gcb,'f32KRs');
      |     f32KLs_bkup=get_param(gcb,'f32KLs');
      |     u16NShift_bkup=get_param(gcb,'u16NShift');
      |     Rs=Simulink.data.evalinGlobal(bdroot,get_param(gcb,'Rs'));
      |     Ls=Simulink.data.evalinGlobal(bdroot,get_param(gcb,'Ls'));
      |     mechspeed=Simulink.data.evalinGlobal(bdroot,get_param(gcb,'mechspeed'));
      |     polepairs=Simulink.data.evalinGlobal(bdroot,get_param(gcb,'polepairs'));
      |     uscale=Simulink.data.evalinGlobal(bdroot,get_param(gcb,'uscale'));
      |     iscale=Simulink.data.evalinGlobal(bdroot,get_param(gcb,'iscale'));
      |     if (Ls<=0)
      |       warning('Inductance Ls must be positive.');
      |     end
      |     if (Rs<0)
      |       warning('Resistance Rs must be non-negative.');
      |     end
      |     if (mechspeed<=0)
      |       warning('Max. speed must be positive.');
      |     end
      |     if (polepairs<1)
      |       warning('Number of pole pairs must be a natural number (1, 2, 3, ...).');
      |     end
      |     if (round(polepairs)~=polepairs)
      |       warning('Number of pole pairs must be a natural number (1, 2, 3, ...).');
      |     end
      |     if (uscale<=0)
      |       warning('U_max must be positive.');
      |     end
      |     if (iscale<=0)
      |       warning('I_max must be positive.');
      |     end
      |     wmax=polepairs*mechspeed*1.047197551196598e-01;
      |     Rssc=Rs*iscale/uscale;
      |     Lssc=Ls*wmax*iscale/uscale;
      |     u16NShift=ceil(log2(abs(Rssc)));
      |     tmpsh=ceil(log2(abs(Lssc)));
      |     if u16NShift<tmpsh
      |       u16NShift=tmpsh;
      |     end
      |     if u16NShift<0
      |       u16NShift=0;
      |     end
      |     if u16NShift>31
      |       u16NShift=31;
      |       warning(['Parameter u16NShift of ' gcb ' exceeds the fixed-point range.']);
      |     end
      |     f32KRs=round(Rssc*2^(-u16NShift)*2^31);
      |     if f32KRs>2^31-1
      |       f32KRs=2^31-1;
      |       warning(['Parameter f32KRs of ' gcb ' exceeds the fixed-point range.']);
      |     end
      |     if f32KRs<-2^31
      |       f32KRs=-2^31;
      |       warning(['Parameter f32KRs of ' gcb ' exceeds the fixed-point range.']);
      |     end
      |     f32KLs=round(Lssc*2^(-u16NShift)*2^31);
      |     if f32KLs>2^31-1
      |       f32KLs=2^31-1;
      |       warning(['Parameter f32KLs of ' gcb ' exceeds the fixed-point range.']);
      |     end
      |     if f32KLs<-2^31
      |       f32KLs=-2^31;
      |       warning(['Parameter f32KLs of ' gcb ' exceeds the fixed-point range.']);
      |     end
      |     if isnan(f32KRs)
      |       if ~strcmp(f32KRs_bkup,'0')
      |         set_param(gcb,'f32KRs','0');
      |       end
      |     else
      |       tmps=num2str(f32KRs);
      |       if ~strcmp(f32KRs_bkup,tmps)
      |         set_param(gcb,'f32KRs',tmps);
      |       end
      |     end
      |     if isnan(f32KLs)
      |       if ~strcmp(f32KLs_bkup,'0')
      |         set_param(gcb,'f32KLs','0');
      |       end
      |     else
      |       tmps=num2str(f32KLs);
      |       if ~strcmp(f32KLs_bkup,tmps)
      |         set_param(gcb,'f32KLs',tmps);
      |       end
      |     end
      |     if isnan(u16NShift)
      |       if ~strcmp(u16NShift_bkup,'0')
      |         set_param(gcb,'u16NShift','0');
      |       end
      |     else
      |       tmps=num2str(u16NShift);
      |       if ~strcmp(u16NShift_bkup,tmps)
      |         set_param(gcb,'u16NShift',tmps);
      |       end
      |     end
      |   else
      |     param=p.getParameter('iscale');
      |     if strcmp(param.Enabled,'on')
      |       p=Simulink.Mask.get(gcb);
      |       param=p.getParameter('Rs');
      |       param.set('Enabled','off');
      |       param=p.getParameter('Ls');
      |       param.set('Enabled','off');
      |       param=p.getParameter('mechspeed');
      |       param.set('Enabled','off');
      |       param=p.getParameter('polepairs');
      |       param.set('Enabled','off');
      |       param=p.getParameter('uscale');
      |       param.set('Enabled','off');
      |       param=p.getParameter('iscale');
      |       param.set('Enabled','off');
      |     end
      |   end
      | end
      mask Display:
      | color('black');
      | pos = get_param(gcb, 'Position');
      | width = pos(3) - pos(1);
      | height = pos(4) - pos(2);
      | tX=width/2;
      | tY=height - 8;
      | color('black');
      | text(tX,tY, 'AMCLIB_FluxEstimAB_F32', 'horizontalAlignment', 'center');
      | if showStates == 2
      |   color('red');
      |   text(tX,tY - 20, ['debugging mode' char(13) char(10) '(limited performance)'], 'horizontalAlignment', 'center');
      | end
  AMCLIB_SpeedLoop_F32 : Subsystem  StartFcn=|  TreatAsAtomicUnit=on  mask(AMCLIB_SpeedLoop_F32){showStates=Hide (faster execution), resetStatesEnable=Pre-set according to the first set of inputs after reset, showDebugOutputs=Hide, f32State_Out_showOutput=off, SampleTime=-1, wf0=30, wksi=1, J=1.6e-5, Kt=0.067, lambdaW=0.9, ramprpm=6, mechspeed=3000, polepairs=1, uscale=15, iscale=10, autoCalcEn=on, u16NSamplesW=0, f32PropGainQ=0, f32IntegGainQ=0, s16PropGainShiftQ=0, s16IntegGainShiftQ=0, f32LowerLimitQ=0, f32UpperLimitQ=0, f32RampUp=0, f32RampDown=0, SampleTime_1=NaN}
      | ts=get_param(gcb,'CompiledSampleTime');
      | if iscell(ts)
      |   ts=ts{1};
      |   if iscell(ts)
      |     ts=ts{1};
      |   end
      | end
      | ts=ts(1);
      | set_param(gcb,'SampleTime_1',num2str(ts));
      | p=Simulink.Mask.get(gcb);
      | hintText=p.getDialogControl('timeHint');
      | SampleTime=Simulink.data.evalinGlobal(bdroot,get_param(gcb,'SampleTime'));
      | p=Simulink.Mask.get(gcb);
      | autoCalcEn=get_param(gcb,'autoCalcEn');
      | if strcmp(autoCalcEn,'on')
      |   if SampleTime==-1
      |     hintText.Prompt='Caution: Implementation parameters depend on inherited sample time. Make sure that the sample time of the block''s inputs corresponds to the sampling period in the target application.';
      |   else
      |     hintText.Prompt='Caution: Implementation parameters depend on the sample time. Make sure that the simulation time step corresponds to the sampling period in the target application.';
      |   end
      |   SampleTime=ts;
      |   u16NSamplesW_bkup=get_param(gcb,'u16NSamplesW');
      |   f32PropGainQ_bkup=get_param(gcb,'f32PropGainQ');
      |   f32IntegGainQ_bkup=get_param(gcb,'f32IntegGainQ');
      |   s16PropGainShiftQ_bkup=get_param(gcb,'s16PropGainShiftQ');
      |   s16IntegGainShiftQ_bkup=get_param(gcb,'s16IntegGainShiftQ');
      |   f32LowerLimitQ_bkup=get_param(gcb,'f32LowerLimitQ');
      |   f32UpperLimitQ_bkup=get_param(gcb,'f32UpperLimitQ');
      |   f32RampUp_bkup=get_param(gcb,'f32RampUp');
      |   f32RampDown_bkup=get_param(gcb,'f32RampDown');
      |   wf0=Simulink.data.evalinGlobal(bdroot,get_param(gcb,'wf0'));
      |   wksi=Simulink.data.evalinGlobal(bdroot,get_param(gcb,'wksi'));
      |   J=Simulink.data.evalinGlobal(bdroot,get_param(gcb,'J'));
      |   Kt=Simulink.data.evalinGlobal(bdroot,get_param(gcb,'Kt'));
      |   lambdaW=Simulink.data.evalinGlobal(bdroot,get_param(gcb,'lambdaW'));
      |   ramprpm=Simulink.data.evalinGlobal(bdroot,get_param(gcb,'ramprpm'));
      |   mechspeed=Simulink.data.evalinGlobal(bdroot,get_param(gcb,'mechspeed'));
      |   polepairs=Simulink.data.evalinGlobal(bdroot,get_param(gcb,'polepairs'));
      |   uscale=Simulink.data.evalinGlobal(bdroot,get_param(gcb,'uscale'));
      |   iscale=Simulink.data.evalinGlobal(bdroot,get_param(gcb,'iscale'));
      |   if (wf0<=0)
      |     warning('Natural frequency f0 must be positive.');
      |   end
      |   if (wksi<=0)
      |     warning('Current loop attenuation must be positive.');
      |   end
      |   if (wksi>1)
      |     warning('Current loop attenuation must not exceed 1.');
      |   end
      |   if (J<=0)
      |     warning('Moment of inertia J must be positive.');
      |   end
      |   if (Kt<=0)
      |     warning('Torque constant Kt must be positive.');
      |   end
      |   if (lambdaW<0)
      |     warning('MA filter smoothing factor must be in the range 0..1.');
      |   end
      |   if (lambdaW>1)
      |     warning('MA filter smoothing factor must be in the range 0..1.');
      |   end
      |   if (mechspeed<=0)
      |     warning('Max. speed must be positive.');
      |   end
      |   if (polepairs<1)
      |     warning('Number of pole pairs must be a natural number (1, 2, 3, ...).');
      |   end
      |   if (round(polepairs)~=polepairs)
      |     warning('Number of pole pairs must be a natural number (1, 2, 3, ...).');
      |   end
      |   if (uscale<=0)
      |     warning('U_max must be positive.');
      |   end
      |   if (iscale<=0)
      |     warning('I_max must be positive.');
      |   end
      |   w0=6.283185307179586*wf0;
      |   pgain=2.0*wksi*w0*J/Kt;
      |   igain=w0*w0*J/Kt;
      |   wmax=polepairs*mechspeed*0.1047197551196598;
      |   kpf=pgain*wmax/iscale;
      |   s16PropGainShiftQ=ceil(log2(abs(kpf)));
      |   if s16PropGainShiftQ<-31
      |     s16PropGainShiftQ=-31;
      |   end
      |   if s16PropGainShiftQ>31
      |     s16PropGainShiftQ=31;
      |     warning(['Parameter s16PropGainShiftQ of ' gcb ' exceeds the fixed-point range.']);
      |   end
      |   f32PropGainQ=round(kpf*2^(-s16PropGainShiftQ)*2^31);
      |   if f32PropGainQ>2^31-1
      |     f32PropGainQ=2^31-1;
      |     warning(['Parameter f32PropGainQ of ' gcb ' exceeds the fixed-point range.']);
      |   end
      |   if f32PropGainQ<-2^31
      |     f32PropGainQ=-2^31;
      |     warning(['Parameter f32PropGainQ of ' gcb ' exceeds the fixed-point range.']);
      |   end
      |   kif=igain*SampleTime*0.5*wmax/iscale;
      |   s16IntegGainShiftQ=ceil(log2(abs(kif)));
      |   if s16IntegGainShiftQ<-31
      |     s16IntegGainShiftQ=-31;
      |   end
      |   if s16IntegGainShiftQ>31
      |     s16IntegGainShiftQ=31;
      |     warning(['Parameter s16IntegGainShiftQ of ' gcb ' exceeds the fixed-point range.']);
      |   end
      |   f32IntegGainQ=round(kif*2^(-s16IntegGainShiftQ)*2^31);
      |   if f32IntegGainQ>2^31-1
      |     f32IntegGainQ=2^31-1;
      |     warning(['Parameter f32IntegGainQ of ' gcb ' exceeds the fixed-point range.']);
      |   end
      |   if f32IntegGainQ<-2^31
      |     f32IntegGainQ=-2^31;
      |     warning(['Parameter f32IntegGainQ of ' gcb ' exceeds the fixed-point range.']);
      |   end
      |   f32LowerLimitQ=-2147483648;
      |   f32UpperLimitQ=2147483647;
      |   u16NSamplesW=round(log2(1.0/abs(lambdaW)));
      |   if u16NSamplesW>31
      |     u16NSamplesW=31;
      |   end
      |   if u16NSamplesW<0
      |     u16NSamplesW=0;
      |   end
      |   rampsc=polepairs*abs(ramprpm)*0.1047197551196598/wmax;
      |   f32RampUp=round(rampsc*2^31);
      |   if f32RampUp>2^31-1
      |     f32RampUp=2^31-1;
      |     warning(['Parameter f32RampUp of ' gcb ' exceeds the fixed-point range.']);
      |   end
      |   if f32RampUp<-2^31
      |     f32RampUp=-2^31;
      |     warning(['Parameter f32RampUp of ' gcb ' exceeds the fixed-point range.']);
      |   end
      |   f32RampDown=round(rampsc*2^31);
      |   if f32RampDown>2^31-1
      |     f32RampDown=2^31-1;
      |     warning(['Parameter f32RampDown of ' gcb ' exceeds the fixed-point range.']);
      |   end
      |   if f32RampDown<-2^31
      |     f32RampDown=-2^31;
      |     warning(['Parameter f32RampDown of ' gcb ' exceeds the fixed-point range.']);
      |   end
      |   if isnan(u16NSamplesW)
      |     if ~strcmp(u16NSamplesW_bkup,'0')
      |       set_param(gcb,'u16NSamplesW','0');
      |     end
      |   else
      |     tmps=num2str(u16NSamplesW);
      |     if ~strcmp(u16NSamplesW_bkup,tmps)
      |       set_param(gcb,'u16NSamplesW',tmps);
      |     end
      |   end
      |   if isnan(f32PropGainQ)
      |     if ~strcmp(f32PropGainQ_bkup,'0')
      |       set_param(gcb,'f32PropGainQ','0');
      |     end
      |   else
      |     tmps=num2str(f32PropGainQ);
      |     if ~strcmp(f32PropGainQ_bkup,tmps)
      |       set_param(gcb,'f32PropGainQ',tmps);
      |     end
      |   end
      |   if isnan(f32IntegGainQ)
      |     if ~strcmp(f32IntegGainQ_bkup,'0')
      |       set_param(gcb,'f32IntegGainQ','0');
      |     end
      |   else
      |     tmps=num2str(f32IntegGainQ);
      |     if ~strcmp(f32IntegGainQ_bkup,tmps)
      |       set_param(gcb,'f32IntegGainQ',tmps);
      |     end
      |   end
      |   if isnan(s16PropGainShiftQ)
      |     if ~strcmp(s16PropGainShiftQ_bkup,'0')
      |       set_param(gcb,'s16PropGainShiftQ','0');
      |     end
      |   else
      |     tmps=num2str(s16PropGainShiftQ);
      |     if ~strcmp(s16PropGainShiftQ_bkup,tmps)
      |       set_param(gcb,'s16PropGainShiftQ',tmps);
      |     end
      |   end
      |   if isnan(s16IntegGainShiftQ)
      |     if ~strcmp(s16IntegGainShiftQ_bkup,'0')
      |       set_param(gcb,'s16IntegGainShiftQ','0');
      |     end
      |   else
      |     tmps=num2str(s16IntegGainShiftQ);
      |     if ~strcmp(s16IntegGainShiftQ_bkup,tmps)
      |       set_param(gcb,'s16IntegGainShiftQ',tmps);
      |     end
      |   end
      |   if isnan(f32LowerLimitQ)
      |     if ~strcmp(f32LowerLimitQ_bkup,'0')
      |       set_param(gcb,'f32LowerLimitQ','0');
      |     end
      |   else
      |     tmps=num2str(f32LowerLimitQ);
      |     if ~strcmp(f32LowerLimitQ_bkup,tmps)
      |       set_param(gcb,'f32LowerLimitQ',tmps);
      |     end
      |   end
      |   if isnan(f32UpperLimitQ)
      |     if ~strcmp(f32UpperLimitQ_bkup,'0')
      |       set_param(gcb,'f32UpperLimitQ','0');
      |     end
      |   else
      |     tmps=num2str(f32UpperLimitQ);
      |     if ~strcmp(f32UpperLimitQ_bkup,tmps)
      |       set_param(gcb,'f32UpperLimitQ',tmps);
      |     end
      |   end
      |   if isnan(f32RampUp)
      |     if ~strcmp(f32RampUp_bkup,'0')
      |       set_param(gcb,'f32RampUp','0');
      |     end
      |   else
      |     tmps=num2str(f32RampUp);
      |     if ~strcmp(f32RampUp_bkup,tmps)
      |       set_param(gcb,'f32RampUp',tmps);
      |     end
      |   end
      |   if isnan(f32RampDown)
      |     if ~strcmp(f32RampDown_bkup,'0')
      |       set_param(gcb,'f32RampDown','0');
      |     end
      |   else
      |     tmps=num2str(f32RampDown);
      |     if ~strcmp(f32RampDown_bkup,tmps)
      |       set_param(gcb,'f32RampDown',tmps);
      |     end
      |   end
      | end
      mask prompts: showStates "Show internal states:"; resetStatesEnable "Internal state after reset:"; showDebugOutputs "Show debugging outputs:"; f32State_Out_showOutput "Output speed ramp state (f32State_Out)"; SampleTime "Sample time (-1 for inherited):"; wf0 "Speed loop natural frequency f0 [Hz]:"; wksi "Speed loop attenuation ξ:"; J "Moment of inertia J [kg*m^2]:"; Kt "Motor torque constant Kt [N*m/A]:"; lambdaW "Speed MA filter smoothing factor λ (0..1):"; ramprpm "Speed ramp slope [ΔRPM per speed loop iteration]:"; mechspeed "Maximum mechanical speed of the motor [RPM]:"; polepairs "Number of pole pairs of the motor:"; uscale "U_max (maximum DC bus voltage) [V]:"; iscale "I_max (maximum phase current) [A]:"; autoCalcEn "Calculate implementation parameters from physical parameters"; u16NSamplesW "u16NSamplesW (GDFLIB_FilterMA - recalculated smoothing factor):"; f32PropGainQ "f32PropGainQ (GFLIB_ControllerPIpAW - proportional gain):"; f32IntegGainQ "f32IntegGainQ (GFLIB_ControllerPIpAW - integral gain):"; s16PropGainShiftQ "s16PropGainShiftQ (GFLIB_ControllerPIpAW - scaling bitwise shift applied to the proportional gain):"; s16IntegGainShiftQ "s16IntegGainShiftQ (GFLIB_ControllerPIpAW - scaling bitwise shift applied to the integral gain):"; f32LowerLimitQ "f32LowerLimitQ (GFLIB_ControllerPIpAW - lower limit):"; f32UpperLimitQ "f32UpperLimitQ (GFLIB_ControllerPIpAW - upper limit):"; f32RampUp "f32RampUp (Ramp up increment coefficient):"; f32RampDown "f32RampDown (Ramp decrement coefficient):"; SampleTime_1 "Discrete sample time:"
      mask help: Speed loop controller for the PMSM field-oriented control algorithm in 32-bit fixed-point fractional implementation. This block supports re-initialization of the internal state during simulation. If the block is reset, the outputs of the MA filter, PI controller, and the ramp will be aligned with the inputs f32FilterMAWOut_preset, f32ControllerPIpAWQOut_preset, and f32RampOut_preset. Refer to the AMMCLIB User's Guide for further details.
      mask init:
      | ddName = get_param(bdroot,'DataDictionary');
      | if length(ddName)==0
      |   set_param(bdroot,'DataDictionary','ammclib_types.sldd');
      | else
      |   dd = Simulink.data.dictionary.open(ddName);
      |   data = getSection(dd,'Design Data');
      |   if ~exist(data,'SWLIBS_2Syst_F16')
      |     addDataSource(dd,'ammclib_types.sldd');
      |     saveChanges(dd);
      |   end
      | end
      | outputsChanged = 0;
      | 
      | if showStates == 1
      |   % hidden state variables
      |   if strcmp(get_param([gcb '/u16NSamplesW'], 'BlockType'), 'Inport')
      |     posblk = get_param(gcb, 'Position');
      | 
      |     pos = get_param([gcb, '/u16NSamplesW'], 'Position');
      |     orient = get_param([gcb, '/u16NSamplesW'], 'Orientation');
      |     delete_block([gcb, '/u16NSamplesW']);
      |     add_block('built-in/Ground', [gcb, '/u16NSamplesW'], 'Position', pos, 'Orientation', orient);
      | 
      |     pos = get_param([gcb, '/f32PropGainQ'], 'Position');
      |     orient = get_param([gcb, '/f32PropGainQ'], 'Orientation');
      |     delete_block([gcb, '/f32PropGainQ']);
      |     add_block('built-in/Ground', [gcb, '/f32PropGainQ'], 'Position', pos, 'Orientation', orient);
      | 
      |     pos = get_param([gcb, '/f32IntegGainQ'], 'Position');
      |     orient = get_param([gcb, '/f32IntegGainQ'], 'Orientation');
      |     delete_block([gcb, '/f32IntegGainQ']);
      |     add_block('built-in/Ground', [gcb, '/f32IntegGainQ'], 'Position', pos, 'Orientation', orient);
      | 
      |     pos = get_param([gcb, '/s16PropGainShiftQ'], 'Position');
      |     orient = get_param([gcb, '/s16PropGainShiftQ'], 'Orientation');
      |     delete_block([gcb, '/s16PropGainShiftQ']);
      |     add_block('built-in/Ground', [gcb, '/s16PropGainShiftQ'], 'Position', pos, 'Orientation', orient);
      | 
      |     pos = get_param([gcb, '/s16IntegGainShiftQ'], 'Position');
      |     orient = get_param([gcb, '/s16IntegGainShiftQ'], 'Orientation');
      |     delete_block([gcb, '/s16IntegGainShiftQ']);
      |     add_block('built-in/Ground', [gcb, '/s16IntegGainShiftQ'], 'Position', pos, 'Orientation', orient);
      | 
      |     pos = get_param([gcb, '/f32LowerLimitQ'], 'Position');
      |     orient = get_param([gcb, '/f32LowerLimitQ'], 'Orientation');
      |     delete_block([gcb, '/f32LowerLimitQ']);
      |     add_block('built-in/Ground', [gcb, '/f32LowerLimitQ'], 'Position', pos, 'Orientation', orient);
      | 
      |     pos = get_param([gcb, '/f32UpperLimitQ'], 'Position');
      |     orient = get_param([gcb, '/f32UpperLimitQ'], 'Orientation');
      |     delete_block([gcb, '/f32UpperLimitQ']);
      |     add_block('built-in/Ground', [gcb, '/f32UpperLimitQ'], 'Position', pos, 'Orientation', orient);
      | 
      |     pos = get_param([gcb, '/f32RampUp'], 'Position');
      |     orient = get_param([gcb, '/f32RampUp'], 'Orientation');
      |     delete_block([gcb, '/f32RampUp']);
      |     add_block('built-in/Ground', [gcb, '/f32RampUp'], 'Position', pos, 'Orientation', orient);
      | 
      |     pos = get_param([gcb, '/f32RampDown'], 'Position');
      |     orient = get_param([gcb, '/f32RampDown'], 'Orientation');
      |     delete_block([gcb, '/f32RampDown']);
      |     add_block('built-in/Ground', [gcb, '/f32RampDown'], 'Position', pos, 'Orientation', orient);
      | 
      |     pos = get_param([gcb, '/f32AccW'], 'Position');
      |     orient = get_param([gcb, '/f32AccW'], 'Orientation');
      |     delete_block([gcb, '/f32AccW']);
      |     add_block('built-in/Ground', [gcb, '/f32AccW'], 'Position', pos, 'Orientation', orient);
      | 
      |     pos = get_param([gcb, '/f32IntegPartK_1Q'], 'Position');
      |     orient = get_param([gcb, '/f32IntegPartK_1Q'], 'Orientation');
      |     delete_block([gcb, '/f32IntegPartK_1Q']);
      |     add_block('built-in/Ground', [gcb, '/f32IntegPartK_1Q'], 'Position', pos, 'Orientation', orient);
      | 
      |     pos = get_param([gcb, '/f32InK_1Q'], 'Position');
      |     orient = get_param([gcb, '/f32InK_1Q'], 'Orientation');
      |     delete_block([gcb, '/f32InK_1Q']);
      |     add_block('built-in/Ground', [gcb, '/f32InK_1Q'], 'Position', pos, 'Orientation', orient);
      | 
      |     pos = get_param([gcb, '/f32State'], 'Position');
      |     orient = get_param([gcb, '/f32State'], 'Orientation');
      |     delete_block([gcb, '/f32State']);
      |     add_block('built-in/Ground', [gcb, '/f32State'], 'Position', pos, 'Orientation', orient);
      | 
      | 
      |     pmask=Simulink.Mask.get(gcb);
      |     pctrl=pmask.getParameter('SampleTime');
      |     pctrl.set('TypeOptions',{'f32VelocityReq/SampleTime','f32VelocityFbck/SampleTime','f32FilterMAWOut_preset/SampleTime','f32ControllerPIpAWQOut_preset/SampleTime','f32RampOut_preset/SampleTime'});
      | 
      |     pos = get_param([gcb '/f32AccW_Out'], 'Position');
      |     orient = get_param([gcb '/f32AccW_Out'], 'Orientation');
      |     delete_block([gcb '/f32AccW_Out']);
      |     add_block('built-in/Terminator', [gcb '/f32AccW_Out'], 'Position', pos, 'Orientation', orient);
      | 
      |     pos = get_param([gcb '/f32IntegPartK_1Q_Out'], 'Position');
      |     orient = get_param([gcb '/f32IntegPartK_1Q_Out'], 'Orientation');
      |     delete_block([gcb '/f32IntegPartK_1Q_Out']);
      |     add_block('built-in/Terminator', [gcb '/f32IntegPartK_1Q_Out'], 'Position', pos, 'Orientation', orient);
      | 
      |     pos = get_param([gcb '/f32InK_1Q_Out'], 'Position');
      |     orient = get_param([gcb '/f32InK_1Q_Out'], 'Orientation');
      |     delete_block([gcb '/f32InK_1Q_Out']);
      |     add_block('built-in/Terminator', [gcb '/f32InK_1Q_Out'], 'Position', pos, 'Orientation', orient);
      | 
      |     if strcmp(get_param([gcb '/f32WReqFilt'], 'BlockType'), 'Outport')
      |       pos = get_param([gcb '/f32WReqFilt'], 'Position');
      |       orient = get_param([gcb '/f32WReqFilt'], 'Orientation');
      |       delete_block([gcb '/f32WReqFilt']);
      |       add_block('built-in/Terminator', [gcb '/f32WReqFilt'], 'Position', pos, 'Orientation', orient);
      | 
      |       pos = get_param([gcb '/f32WErr'], 'Position');
      |       orient = get_param([gcb '/f32WErr'], 'Orientation');
      |       delete_block([gcb '/f32WErr']);
      |       add_block('built-in/Terminator', [gcb '/f32WErr'], 'Position', pos, 'Orientation', orient);
      | 
      |       pos = get_param([gcb '/f32WFbckFilt'], 'Position');
      |       orient = get_param([gcb '/f32WFbckFilt'], 'Orientation');
      |       delete_block([gcb '/f32WFbckFilt']);
      |       add_block('built-in/Terminator', [gcb '/f32WFbckFilt'], 'Position', pos, 'Orientation', orient);
      | 
      |     end
      | 
      |     set_param([gcb '/f32VelocityReq'], 'Port', '1');
      |     set_param([gcb '/f32VelocityFbck'], 'Port', '2');
      |     set_param([gcb '/f32FilterMAWOut_preset'], 'Port', '3');
      |     set_param([gcb '/f32ControllerPIpAWQOut_preset'], 'Port', '4');
      |     set_param([gcb '/f32RampOut_preset'], 'Port', '5');
      | 
      |     tmpOutCnt=0;
      |     tmpOutCnt=tmpOutCnt+1;
      |     set_param([gcb '/pIDQReq'], 'Port', num2str(tmpOutCnt));
      |     tmpOutCnt=tmpOutCnt+1;
      |     set_param([gcb '/u16LimitFlagQ'], 'Port', num2str(tmpOutCnt));
      |     if strcmp(get_param([gcb '/f32State_Out'], 'BlockType'), 'Outport')
      |       tmpOutCnt=tmpOutCnt+1;
      |       set_param([gcb '/f32State_Out'], 'Port', num2str(tmpOutCnt));
      |     end
      | 
      |   autoCalcEn=get_param(gcb,'autoCalcEn');
      |   if strcmp(autoCalcEn,'on')
      |     set_param(gcb,'MaskEnables',{'on','on','off','on','on','on','on','on','on','on','on','on','on','on','on','on','on','on','on','on','on','on','on','on','on','off'});
      |   else
      |     set_param(gcb,'MaskEnables',{'on','on','off','on','on','off','off','off','off','off','off','off','off','off','off','on','on','on','on','on','on','on','on','on','on','off'});
      |   end
      | 
      |     if (posblk(4) - posblk(2)) > 150
      |       height = 150;
      |       set_param(gcb,'Position',[posblk(1), posblk(2), posblk(3), posblk(2)+height])
      |     end
      |   end
      | else
      |   % shown state variables
      |   if strcmp(get_param([gcb '/u16NSamplesW'], 'BlockType'), 'Ground')
      |     posblk = get_param(gcb, 'Position');
      | 
      |     pos = get_param([gcb, '/u16NSamplesW'], 'Position');
      |     orient = get_param([gcb, '/u16NSamplesW'], 'Orientation');
      |     delete_block([gcb, '/u16NSamplesW']);
      |     add_block('built-in/Inport', [gcb, '/u16NSamplesW'], 'Position', pos, 'Orientation', orient, 'OutDataTypeStr', 'uint16');
      | 
      |     pos = get_param([gcb, '/f32PropGainQ'], 'Position');
      |     orient = get_param([gcb, '/f32PropGainQ'], 'Orientation');
      |     delete_block([gcb, '/f32PropGainQ']);
      |     add_block('built-in/Inport', [gcb, '/f32PropGainQ'], 'Position', pos, 'Orientation', orient, 'OutDataTypeStr', 'int32');
      | 
      |     pos = get_param([gcb, '/f32IntegGainQ'], 'Position');
      |     orient = get_param([gcb, '/f32IntegGainQ'], 'Orientation');
      |     delete_block([gcb, '/f32IntegGainQ']);
      |     add_block('built-in/Inport', [gcb, '/f32IntegGainQ'], 'Position', pos, 'Orientation', orient, 'OutDataTypeStr', 'int32');
      | 
      |     pos = get_param([gcb, '/s16PropGainShiftQ'], 'Position');
      |     orient = get_param([gcb, '/s16PropGainShiftQ'], 'Orientation');
      |     delete_block([gcb, '/s16PropGainShiftQ']);
      |     add_block('built-in/Inport', [gcb, '/s16PropGainShiftQ'], 'Position', pos, 'Orientation', orient, 'OutDataTypeStr', 'int16');
      | 
      |     pos = get_param([gcb, '/s16IntegGainShiftQ'], 'Position');
      |     orient = get_param([gcb, '/s16IntegGainShiftQ'], 'Orientation');
      |     delete_block([gcb, '/s16IntegGainShiftQ']);
      |     add_block('built-in/Inport', [gcb, '/s16IntegGainShiftQ'], 'Position', pos, 'Orientation', orient, 'OutDataTypeStr', 'int16');
      | 
      |     pos = get_param([gcb, '/f32LowerLimitQ'], 'Position');
      |     orient = get_param([gcb, '/f32LowerLimitQ'], 'Orientation');
      |     delete_block([gcb, '/f32LowerLimitQ']);
      |     add_block('built-in/Inport', [gcb, '/f32LowerLimitQ'], 'Position', pos, 'Orientation', orient, 'OutDataTypeStr', 'int32');
      | 
      |     pos = get_param([gcb, '/f32UpperLimitQ'], 'Position');
      |     orient = get_param([gcb, '/f32UpperLimitQ'], 'Orientation');
      |     delete_block([gcb, '/f32UpperLimitQ']);
      |     add_block('built-in/Inport', [gcb, '/f32UpperLimitQ'], 'Position', pos, 'Orientation', orient, 'OutDataTypeStr', 'int32');
      | 
      |     pos = get_param([gcb, '/f32RampUp'], 'Position');
      |     orient = get_param([gcb, '/f32RampUp'], 'Orientation');
      |     delete_block([gcb, '/f32RampUp']);
      |     add_block('built-in/Inport', [gcb, '/f32RampUp'], 'Position', pos, 'Orientation', orient, 'OutDataTypeStr', 'int32');
      | 
      |     pos = get_param([gcb, '/f32RampDown'], 'Position');
      |     orient = get_param([gcb, '/f32RampDown'], 'Orientation');
      |     delete_block([gcb, '/f32RampDown']);
      |     add_block('built-in/Inport', [gcb, '/f32RampDown'], 'Position', pos, 'Orientation', orient, 'OutDataTypeStr', 'int32');
      | 
      |     pos = get_param([gcb, '/f32AccW'], 'Position');
      |     orient = get_param([gcb, '/f32AccW'], 'Orientation');
      |     delete_block([gcb, '/f32AccW']);
      |     add_block('built-in/Inport', [gcb, '/f32AccW'], 'Position', pos, 'Orientation', orient, 'OutDataTypeStr', 'int32');
      | 
      |     pos = get_param([gcb, '/f32IntegPartK_1Q'], 'Position');
      |     orient = get_param([gcb, '/f32IntegPartK_1Q'], 'Orientation');
      |     delete_block([gcb, '/f32IntegPartK_1Q']);
      |     add_block('built-in/Inport', [gcb, '/f32IntegPartK_1Q'], 'Position', pos, 'Orientation', orient, 'OutDataTypeStr', 'int32');
      | 
      |     pos = get_param([gcb, '/f32InK_1Q'], 'Position');
      |     orient = get_param([gcb, '/f32InK_1Q'], 'Orientation');
      |     delete_block([gcb, '/f32InK_1Q']);
      |     add_block('built-in/Inport', [gcb, '/f32InK_1Q'], 'Position', pos, 'Orientation', orient, 'OutDataTypeStr', 'int32');
      | 
      |     pos = get_param([gcb, '/f32State'], 'Position');
      |     orient = get_param([gcb, '/f32State'], 'Orientation');
      |     delete_block([gcb, '/f32State']);
      |     add_block('built-in/Inport', [gcb, '/f32State'], 'Position', pos, 'Orientation', orient, 'OutDataTypeStr', 'int32');
      | 
      | 
      | 
      |     pos = get_param([gcb '/f32AccW_Out'], 'Position');
      |     orient = get_param([gcb '/f32AccW_Out'], 'Orientation');
      |     delete_block([gcb '/f32AccW_Out']);
      |     add_block('built-in/Outport', [gcb '/f32AccW_Out'], 'Position', pos, 'Orientation', orient);
      | 
      |     pos = get_param([gcb '/f32IntegPartK_1Q_Out'], 'Position');
      |     orient = get_param([gcb '/f32IntegPartK_1Q_Out'], 'Orientation');
      |     delete_block([gcb '/f32IntegPartK_1Q_Out']);
      |     add_block('built-in/Outport', [gcb '/f32IntegPartK_1Q_Out'], 'Position', pos, 'Orientation', orient);
      | 
      |     pos = get_param([gcb '/f32InK_1Q_Out'], 'Position');
      |     orient = get_param([gcb '/f32InK_1Q_Out'], 'Orientation');
      |     delete_block([gcb '/f32InK_1Q_Out']);
      |     add_block('built-in/Outport', [gcb '/f32InK_1Q_Out'], 'Position', pos, 'Orientation', orient);
      | 
      | 
      |     pmask=Simulink.Mask.get(gcb);
      |     pctrl=pmask.getParameter('SampleTime');
      |     pctrl.set('TypeOptions',{'f32VelocityReq/SampleTime','f32VelocityFbck/SampleTime','f32FilterMAWOut_preset/SampleTime','f32ControllerPIpAWQOut_preset/SampleTime','f32RampOut_preset/SampleTime','u16NSamplesW/SampleTime','f32PropGainQ/SampleTime','f32IntegGainQ/SampleTime','s16PropGainShiftQ/SampleTime','s16IntegGainShiftQ/SampleTime','f32LowerLimitQ/SampleTime','f32UpperLimitQ/SampleTime','f32RampUp/SampleTime','f32RampDown/SampleTime','f32AccW/SampleTime','f32IntegPartK_1Q/SampleTime','f32InK_1Q/SampleTime','f32State/SampleTime'});
      | 
      |     if (showDebugOutputs == 2) && (strcmp(get_param([gcb '/f32WReqFilt'], 'BlockType'), 'Terminator'))
      |       pos = get_param([gcb '/f32WReqFilt'], 'Position');
      |       orient = get_param([gcb '/f32WReqFilt'], 'Orientation');
      |       delete_block([gcb '/f32WReqFilt']);
      |       add_block('built-in/Outport', [gcb '/f32WReqFilt'], 'Position', pos, 'Orientation', orient);
      | 
      |       pos = get_param([gcb '/f32WErr'], 'Position');
      |       orient = get_param([gcb '/f32WErr'], 'Orientation');
      |       delete_block([gcb '/f32WErr']);
      |       add_block('built-in/Outport', [gcb '/f32WErr'], 'Position', pos, 'Orientation', orient);
      | 
      |       pos = get_param([gcb '/f32WFbckFilt'], 'Position');
      |       orient = get_param([gcb '/f32WFbckFilt'], 'Orientation');
      |       delete_block([gcb '/f32WFbckFilt']);
      |       add_block('built-in/Outport', [gcb '/f32WFbckFilt'], 'Position', pos, 'Orientation', orient);
      | 
      |     end
      | 
      |     set_param([gcb '/f32VelocityReq'], 'Port', '1');
      |     set_param([gcb '/f32VelocityFbck'], 'Port', '2');
      |     set_param([gcb '/f32FilterMAWOut_preset'], 'Port', '3');
      |     set_param([gcb '/f32ControllerPIpAWQOut_preset'], 'Port', '4');
      |     set_param([gcb '/f32RampOut_preset'], 'Port', '5');
      |     set_param([gcb '/u16NSamplesW'], 'Port', '6');
      |     set_param([gcb '/f32PropGainQ'], 'Port', '7');
      |     set_param([gcb '/f32IntegGainQ'], 'Port', '8');
      |     set_param([gcb '/s16PropGainShiftQ'], 'Port', '9');
      |     set_param([gcb '/s16IntegGainShiftQ'], 'Port', '10');
      |     set_param([gcb '/f32LowerLimitQ'], 'Port', '11');
      |     set_param([gcb '/f32UpperLimitQ'], 'Port', '12');
      |     set_param([gcb '/f32RampUp'], 'Port', '13');
      |     set_param([gcb '/f32RampDown'], 'Port', '14');
      |     set_param([gcb '/f32AccW'], 'Port', '15');
      |     set_param([gcb '/f32IntegPartK_1Q'], 'Port', '16');
      |     set_param([gcb '/f32InK_1Q'], 'Port', '17');
      |     set_param([gcb '/f32State'], 'Port', '18');
      | 
      |     if (showDebugOutputs == 2)
      |       tmpOutCnt=0;
      |       tmpOutCnt=tmpOutCnt+1;
      |       set_param([gcb '/pIDQReq'], 'Port', num2str(tmpOutCnt));
      |       tmpOutCnt=tmpOutCnt+1;
      |       set_param([gcb '/u16LimitFlagQ'], 'Port', num2str(tmpOutCnt));
      |       tmpOutCnt=tmpOutCnt+1;
      |       set_param([gcb '/f32WReqFilt'], 'Port', num2str(tmpOutCnt));
      |       tmpOutCnt=tmpOutCnt+1;
      |       set_param([gcb '/f32WErr'], 'Port', num2str(tmpOutCnt));
      |       tmpOutCnt=tmpOutCnt+1;
      |       set_param([gcb '/f32WFbckFilt'], 'Port', num2str(tmpOutCnt));
      |       tmpOutCnt=tmpOutCnt+1;
      |       set_param([gcb '/f32AccW_Out'], 'Port', num2str(tmpOutCnt));
      |       tmpOutCnt=tmpOutCnt+1;
      |       set_param([gcb '/f32IntegPartK_1Q_Out'], 'Port', num2str(tmpOutCnt));
      |       tmpOutCnt=tmpOutCnt+1;
      |       set_param([gcb '/f32InK_1Q_Out'], 'Port', num2str(tmpOutCnt));
      |       if strcmp(get_param([gcb '/f32State_Out'], 'BlockType'), 'Outport')
      |         tmpOutCnt=tmpOutCnt+1;
      |         set_param([gcb '/f32State_Out'], 'Port', num2str(tmpOutCnt));
      |       end
      |     else
      |       tmpOutCnt=0;
      |       tmpOutCnt=tmpOutCnt+1;
      |       set_param([gcb '/pIDQReq'], 'Port', num2str(tmpOutCnt));
      |       tmpOutCnt=tmpOutCnt+1;
      |       set_param([gcb '/u16LimitFlagQ'], 'Port', num2str(tmpOutCnt));
      |       tmpOutCnt=tmpOutCnt+1;
      |       set_param([gcb '/f32AccW_Out'], 'Port', num2str(tmpOutCnt));
      |       tmpOutCnt=tmpOutCnt+1;
      |       set_param([gcb '/f32IntegPartK_1Q_Out'], 'Port', num2str(tmpOutCnt));
      |       tmpOutCnt=tmpOutCnt+1;
      |       set_param([gcb '/f32InK_1Q_Out'], 'Port', num2str(tmpOutCnt));
      |       if strcmp(get_param([gcb '/f32State_Out'], 'BlockType'), 'Outport')
      |         tmpOutCnt=tmpOutCnt+1;
      |         set_param([gcb '/f32State_Out'], 'Port', num2str(tmpOutCnt));
      |       end
      |     end
      | 
      |     set_param(gcb,'MaskEnables',{'on','on','on','on','on','off','off','off','off','off','off','off','off','off','off','off','off','off','off','off','off','off','off','off','off','off'});
      | 
      |     if (posblk(4) - posblk(2)) < 475
      |       height = 475;
      |       set_param(gcb,'Position',[posblk(1), posblk(2), posblk(3), posblk(2)+height])
      |     end
      |   else
      |     if (showDebugOutputs == 2) && (strcmp(get_param([gcb '/f32WReqFilt'], 'BlockType'), 'Terminator'))
      |       % shown debugging outputs
      |       pos = get_param([gcb '/f32WReqFilt'], 'Position');
      |       orient = get_param([gcb '/f32WReqFilt'], 'Orientation');
      |       delete_block([gcb '/f32WReqFilt']);
      |       add_block('built-in/Outport', [gcb '/f32WReqFilt'], 'Position', pos, 'Orientation', orient);
      | 
      |       pos = get_param([gcb '/f32WErr'], 'Position');
      |       orient = get_param([gcb '/f32WErr'], 'Orientation');
      |       delete_block([gcb '/f32WErr']);
      |       add_block('built-in/Outport', [gcb '/f32WErr'], 'Position', pos, 'Orientation', orient);
      | 
      |       pos = get_param([gcb '/f32WFbckFilt'], 'Position');
      |       orient = get_param([gcb '/f32WFbckFilt'], 'Orientation');
      |       delete_block([gcb '/f32WFbckFilt']);
      |       add_block('built-in/Outport', [gcb '/f32WFbckFilt'], 'Position', pos, 'Orientation', orient);
      | 
      |       tmpOutCnt=0;
      |       tmpOutCnt=tmpOutCnt+1;
      |       set_param([gcb '/pIDQReq'], 'Port', num2str(tmpOutCnt));
      |       tmpOutCnt=tmpOutCnt+1;
      |       set_param([gcb '/u16LimitFlagQ'], 'Port', num2str(tmpOutCnt));
      |       tmpOutCnt=tmpOutCnt+1;
      |       set_param([gcb '/f32WReqFilt'], 'Port', num2str(tmpOutCnt));
      |       tmpOutCnt=tmpOutCnt+1;
      |       set_param([gcb '/f32WErr'], 'Port', num2str(tmpOutCnt));
      |       tmpOutCnt=tmpOutCnt+1;
      |       set_param([gcb '/f32WFbckFilt'], 'Port', num2str(tmpOutCnt));
      |       tmpOutCnt=tmpOutCnt+1;
      |       set_param([gcb '/f32AccW_Out'], 'Port', num2str(tmpOutCnt));
      |       tmpOutCnt=tmpOutCnt+1;
      |       set_param([gcb '/f32IntegPartK_1Q_Out'], 'Port', num2str(tmpOutCnt));
      |       tmpOutCnt=tmpOutCnt+1;
      |       set_param([gcb '/f32InK_1Q_Out'], 'Port', num2str(tmpOutCnt));
      |       if strcmp(get_param([gcb '/f32State_Out'], 'BlockType'), 'Outport')
      |         tmpOutCnt=tmpOutCnt+1;
      |         set_param([gcb '/f32State_Out'], 'Port', num2str(tmpOutCnt));
      |       end
      |     elseif (showDebugOutputs == 1) && (strcmp(get_param([gcb '/f32WReqFilt'], 'BlockType'), 'Outport'))
      |       % hidden debugging outputs
      |       pos = get_param([gcb '/f32WReqFilt'], 'Position');
      |       orient = get_param([gcb '/f32WReqFilt'], 'Orientation');
      |       delete_block([gcb '/f32WReqFilt']);
      |       add_block('built-in/Terminator', [gcb '/f32WReqFilt'], 'Position', pos, 'Orientation', orient);
      | 
      |       pos = get_param([gcb '/f32WErr'], 'Position');
      |       orient = get_param([gcb '/f32WErr'], 'Orientation');
      |       delete_block([gcb '/f32WErr']);
      |       add_block('built-in/Terminator', [gcb '/f32WErr'], 'Position', pos, 'Orientation', orient);
      | 
      |       pos = get_param([gcb '/f32WFbckFilt'], 'Position');
      |       orient = get_param([gcb '/f32WFbckFilt'], 'Orientation');
      |       delete_block([gcb '/f32WFbckFilt']);
      |       add_block('built-in/Terminator', [gcb '/f32WFbckFilt'], 'Position', pos, 'Orientation', orient);
      | 
      |       tmpOutCnt=0;
      |       tmpOutCnt=tmpOutCnt+1;
      |       set_param([gcb '/pIDQReq'], 'Port', num2str(tmpOutCnt));
      |       tmpOutCnt=tmpOutCnt+1;
      |       set_param([gcb '/u16LimitFlagQ'], 'Port', num2str(tmpOutCnt));
      |       tmpOutCnt=tmpOutCnt+1;
      |       set_param([gcb '/f32AccW_Out'], 'Port', num2str(tmpOutCnt));
      |       tmpOutCnt=tmpOutCnt+1;
      |       set_param([gcb '/f32IntegPartK_1Q_Out'], 'Port', num2str(tmpOutCnt));
      |       tmpOutCnt=tmpOutCnt+1;
      |       set_param([gcb '/f32InK_1Q_Out'], 'Port', num2str(tmpOutCnt));
      |       if strcmp(get_param([gcb '/f32State_Out'], 'BlockType'), 'Outport')
      |         tmpOutCnt=tmpOutCnt+1;
      |         set_param([gcb '/f32State_Out'], 'Port', num2str(tmpOutCnt));
      |       end
      |     end
      |   end
      | end
      | if strcmp(get_param(gcb,'f32State_Out_showOutput'),'on')
      |   if strcmp(get_param([gcb '/f32State_Out'], 'BlockType'), 'Terminator')
      |     pos = get_param([gcb '/f32State_Out'], 'Position');
      |     orient = get_param([gcb '/f32State_Out'], 'Orientation');
      |     delete_block([gcb '/f32State_Out']);
      |     add_block('built-in/Outport', [gcb '/f32State_Out'], 'Position', pos, 'Orientation', orient);
      |     outputsChanged = 1;
      |   end
      | else
      |   if strcmp(get_param([gcb '/f32State_Out'], 'BlockType'), 'Outport')
      |     pos = get_param([gcb '/f32State_Out'], 'Position');
      |     orient = get_param([gcb '/f32State_Out'], 'Orientation');
      |     delete_block([gcb '/f32State_Out']);
      |     add_block('built-in/Terminator', [gcb '/f32State_Out'], 'Position', pos, 'Orientation', orient);
      |     outputsChanged = 1;
      |   end
      | end
      | if outputsChanged == 1;
      |   tmpOutCnt = 0;
      |   if strcmp(get_param([gcb '/pIDQReq'], 'BlockType'), 'Outport')
      |     tmpOutCnt = tmpOutCnt + 1;
      |     set_param([gcb '/pIDQReq'], 'Port', num2str(tmpOutCnt));
      |   end
      |   if strcmp(get_param([gcb '/u16LimitFlagQ'], 'BlockType'), 'Outport')
      |     tmpOutCnt = tmpOutCnt + 1;
      |     set_param([gcb '/u16LimitFlagQ'], 'Port', num2str(tmpOutCnt));
      |   end
      |   if strcmp(get_param([gcb '/f32WReqFilt'], 'BlockType'), 'Outport')
      |     tmpOutCnt = tmpOutCnt + 1;
      |     set_param([gcb '/f32WReqFilt'], 'Port', num2str(tmpOutCnt));
      |   end
      |   if strcmp(get_param([gcb '/f32WErr'], 'BlockType'), 'Outport')
      |     tmpOutCnt = tmpOutCnt + 1;
      |     set_param([gcb '/f32WErr'], 'Port', num2str(tmpOutCnt));
      |   end
      |   if strcmp(get_param([gcb '/f32WFbckFilt'], 'BlockType'), 'Outport')
      |     tmpOutCnt = tmpOutCnt + 1;
      |     set_param([gcb '/f32WFbckFilt'], 'Port', num2str(tmpOutCnt));
      |   end
      |   if strcmp(get_param([gcb '/f32AccW_Out'], 'BlockType'), 'Outport')
      |     tmpOutCnt = tmpOutCnt + 1;
      |     set_param([gcb '/f32AccW_Out'], 'Port', num2str(tmpOutCnt));
      |   end
      |   if strcmp(get_param([gcb '/f32IntegPartK_1Q_Out'], 'BlockType'), 'Outport')
      |     tmpOutCnt = tmpOutCnt + 1;
      |     set_param([gcb '/f32IntegPartK_1Q_Out'], 'Port', num2str(tmpOutCnt));
      |   end
      |   if strcmp(get_param([gcb '/f32InK_1Q_Out'], 'BlockType'), 'Outport')
      |     tmpOutCnt = tmpOutCnt + 1;
      |     set_param([gcb '/f32InK_1Q_Out'], 'Port', num2str(tmpOutCnt));
      |   end
      |   if strcmp(get_param([gcb '/f32State_Out'], 'BlockType'), 'Outport')
      |     tmpOutCnt = tmpOutCnt + 1;
      |     set_param([gcb '/f32State_Out'], 'Port', num2str(tmpOutCnt));
      |   end
      | end
      settings: RTWSystemCode=Inline
      mask Help: web([fileparts(which('ammclib_bam_S32K3xx.slx')) '/../doc/S32K3XXMCLUG.pdf'], '-browser')
      mask TypeOptions showStates: Hide (faster execution) | Show (allows debugging; connect feedback loops manually)
      mask Callback showStates:
      | maskStr=get_param(gcb,'showStates');
      | if strcmp(maskStr,'Hide (faster execution)')
      |   autoCalcEn=get_param(gcb,'autoCalcEn');
      |   if strcmp(autoCalcEn,'on')
      |     set_param(gcb,'MaskEnables',{'on','on','off','on','on','on','on','on','on','on','on','on','on','on','on','on','on','on','on','on','on','on','on','on','on','off'});
      |   else
      |     set_param(gcb,'MaskEnables',{'on','on','off','on','on','off','off','off','off','off','off','off','off','off','off','on','on','on','on','on','on','on','on','on','on','off'});
      |   end
      | else
      |   set_param(gcb,'MaskEnables',{'on','on','on','on','on','off','off','off','off','off','off','off','off','off','off','off','off','off','off','off','off','off','off','off','off','off'});
      | end
      mask TypeOptions resetStatesEnable: Pre-set according to the first set of inputs after reset | Clear to zero
      mask TypeOptions showDebugOutputs: Hide | Show
      mask TypeOptions SampleTime: f32VelocityReq/SampleTime | f32VelocityFbck/SampleTime | f32FilterMAWOut_preset/SampleTime | f32ControllerPIpAWQOut_preset/SampleTime | f32RampOut_preset/SampleTime
      mask Callback SampleTime:
      | p=Simulink.Mask.get(gcb);
      | hintText=p.getDialogControl('timeHint');
      | SampleTime=Simulink.data.evalinGlobal(bdroot,get_param(gcb,'SampleTime'));
      | SampleTime_1=str2double(get_param(gcb,'SampleTime_1'));
      | if (((SampleTime==-1) && (~contains(hintText.Prompt,'inherited'))) || ...
      |     ((SampleTime~=-1) && contains(hintText.Prompt,'inherited')) || ...
      |     ((SampleTime~=-1) && (SampleTime_1~=SampleTime)) || ...
      |     ((SampleTime_1~=-1) && contains(hintText.Prompt,'yet')))
      |   if ((SampleTime==-1) && (~contains(hintText.Prompt,'inherited')))
      |     set_param(gcb,'SampleTime_1',num2str(NaN));
      |     SampleTime_1=NaN;
      |   end
      |   if (SampleTime~=-1)
      |     set_param(gcb,'SampleTime_1',num2str(SampleTime));
      |     SampleTime_1=SampleTime;
      |   end
      |   autoCalcEn=get_param(gcb,'autoCalcEn');
      |   if strcmp(autoCalcEn,'on')
      |     p=Simulink.Mask.get(gcb);
      |     hintText=p.getDialogControl('timeHint');
      |     if SampleTime==-1
      |       SampleTime=SampleTime_1;
      |       if isnan(SampleTime)
      |         hintText.Prompt='Note: Implementation parameters cannot be calculated yet because the block''s inherited sample time is unknown. Simulink will update the sample time when you run the simulation.';
      |       else
      |         hintText.Prompt='Caution: Implementation parameters depend on inherited sample time. Make sure that the sample time of the block''s inputs corresponds to the sampling period in the target application.';
      |       end
      |     else
      |       hintText.Prompt='Caution: Implementation parameters depend on the sample time. Make sure that the simulation time step corresponds to the sampling period in the target application.';
      |     end
      |     u16NSamplesW_bkup=get_param(gcb,'u16NSamplesW');
      |     f32PropGainQ_bkup=get_param(gcb,'f32PropGainQ');
      |     f32IntegGainQ_bkup=get_param(gcb,'f32IntegGainQ');
      |     s16PropGainShiftQ_bkup=get_param(gcb,'s16PropGainShiftQ');
      |     s16IntegGainShiftQ_bkup=get_param(gcb,'s16IntegGainShiftQ');
      |     f32LowerLimitQ_bkup=get_param(gcb,'f32LowerLimitQ');
      |     f32UpperLimitQ_bkup=get_param(gcb,'f32UpperLimitQ');
      |     f32RampUp_bkup=get_param(gcb,'f32RampUp');
      |     f32RampDown_bkup=get_param(gcb,'f32RampDown');
      |     wf0=Simulink.data.evalinGlobal(bdroot,get_param(gcb,'wf0'));
      |     wksi=Simulink.data.evalinGlobal(bdroot,get_param(gcb,'wksi'));
      |     J=Simulink.data.evalinGlobal(bdroot,get_param(gcb,'J'));
      |     Kt=Simulink.data.evalinGlobal(bdroot,get_param(gcb,'Kt'));
      |     lambdaW=Simulink.data.evalinGlobal(bdroot,get_param(gcb,'lambdaW'));
      |     ramprpm=Simulink.data.evalinGlobal(bdroot,get_param(gcb,'ramprpm'));
      |     mechspeed=Simulink.data.evalinGlobal(bdroot,get_param(gcb,'mechspeed'));
      |     polepairs=Simulink.data.evalinGlobal(bdroot,get_param(gcb,'polepairs'));
      |     uscale=Simulink.data.evalinGlobal(bdroot,get_param(gcb,'uscale'));
      |     iscale=Simulink.data.evalinGlobal(bdroot,get_param(gcb,'iscale'));
      |     if (wf0<=0)
      |       warning('Natural frequency f0 must be positive.');
      |     end
      |     if (wksi<=0)
      |       warning('Current loop attenuation must be positive.');
      |     end
      |     if (wksi>1)
      |       warning('Current loop attenuation must not exceed 1.');
      |     end
      |     if (J<=0)
      |       warning('Moment of inertia J must be positive.');
      |     end
      |     if (Kt<=0)
      |       warning('Torque constant Kt must be positive.');
      |     end
      |     if (lambdaW<0)
      |       warning('MA filter smoothing factor must be in the range 0..1.');
      |     end
      |     if (lambdaW>1)
      |       warning('MA filter smoothing factor must be in the range 0..1.');
      |     end
      |     if (mechspeed<=0)
      |       warning('Max. speed must be positive.');
      |     end
      |     if (polepairs<1)
      |       warning('Number of pole pairs must be a natural number (1, 2, 3, ...).');
      |     end
      |     if (round(polepairs)~=polepairs)
      |       warning('Number of pole pairs must be a natural number (1, 2, 3, ...).');
      |     end
      |     if (uscale<=0)
      |       warning('U_max must be positive.');
      |     end
      |     if (iscale<=0)
      |       warning('I_max must be positive.');
      |     end
      |     w0=6.283185307179586*wf0;
      |     pgain=2.0*wksi*w0*J/Kt;
      |     igain=w0*w0*J/Kt;
      |     wmax=polepairs*mechspeed*0.1047197551196598;
      |     kpf=pgain*wmax/iscale;
      |     s16PropGainShiftQ=ceil(log2(abs(kpf)));
      |     if s16PropGainShiftQ<-31
      |       s16PropGainShiftQ=-31;
      |     end
      |     if s16PropGainShiftQ>31
      |       s16PropGainShiftQ=31;
      |       warning(['Parameter s16PropGainShiftQ of ' gcb ' exceeds the fixed-point range.']);
      |     end
      |     f32PropGainQ=round(kpf*2^(-s16PropGainShiftQ)*2^31);
      |     if f32PropGainQ>2^31-1
      |       f32PropGainQ=2^31-1;
      |       warning(['Parameter f32PropGainQ of ' gcb ' exceeds the fixed-point range.']);
      |     end
      |     if f32PropGainQ<-2^31
      |       f32PropGainQ=-2^31;
      |       warning(['Parameter f32PropGainQ of ' gcb ' exceeds the fixed-point range.']);
      |     end
      |     kif=igain*SampleTime*0.5*wmax/iscale;
      |     s16IntegGainShiftQ=ceil(log2(abs(kif)));
      |     if s16IntegGainShiftQ<-31
      |       s16IntegGainShiftQ=-31;
      |     end
      |     if s16IntegGainShiftQ>31
      |       s16IntegGainShiftQ=31;
      |       warning(['Parameter s16IntegGainShiftQ of ' gcb ' exceeds the fixed-point range.']);
      |     end
      |     f32IntegGainQ=round(kif*2^(-s16IntegGainShiftQ)*2^31);
      |     if f32IntegGainQ>2^31-1
      |       f32IntegGainQ=2^31-1;
      |       warning(['Parameter f32IntegGainQ of ' gcb ' exceeds the fixed-point range.']);
      |     end
      |     if f32IntegGainQ<-2^31
      |       f32IntegGainQ=-2^31;
      |       warning(['Parameter f32IntegGainQ of ' gcb ' exceeds the fixed-point range.']);
      |     end
      |     f32LowerLimitQ=-2147483648;
      |     f32UpperLimitQ=2147483647;
      |     u16NSamplesW=round(log2(1.0/abs(lambdaW)));
      |     if u16NSamplesW>31
      |       u16NSamplesW=31;
      |     end
      |     if u16NSamplesW<0
      |       u16NSamplesW=0;
      |     end
      |     rampsc=polepairs*abs(ramprpm)*0.1047197551196598/wmax;
      |     f32RampUp=round(rampsc*2^31);
      |     if f32RampUp>2^31-1
      |       f32RampUp=2^31-1;
      |       warning(['Parameter f32RampUp of ' gcb ' exceeds the fixed-point range.']);
      |     end
      |     if f32RampUp<-2^31
      |       f32RampUp=-2^31;
      |       warning(['Parameter f32RampUp of ' gcb ' exceeds the fixed-point range.']);
      |     end
      |     f32RampDown=round(rampsc*2^31);
      |     if f32RampDown>2^31-1
      |       f32RampDown=2^31-1;
      |       warning(['Parameter f32RampDown of ' gcb ' exceeds the fixed-point range.']);
      |     end
      |     if f32RampDown<-2^31
      |       f32RampDown=-2^31;
      |       warning(['Parameter f32RampDown of ' gcb ' exceeds the fixed-point range.']);
      |     end
      |     if isnan(u16NSamplesW)
      |       if ~strcmp(u16NSamplesW_bkup,'0')
      |         set_param(gcb,'u16NSamplesW','0');
      |       end
      |     else
      |       tmps=num2str(u16NSamplesW);
      |       if ~strcmp(u16NSamplesW_bkup,tmps)
      |         set_param(gcb,'u16NSamplesW',tmps);
      |       end
      |     end
      |     if isnan(f32PropGainQ)
      |       if ~strcmp(f32PropGainQ_bkup,'0')
      |         set_param(gcb,'f32PropGainQ','0');
      |       end
      |     else
      |       tmps=num2str(f32PropGainQ);
      |       if ~strcmp(f32PropGainQ_bkup,tmps)
      |         set_param(gcb,'f32PropGainQ',tmps);
      |       end
      |     end
      |     if isnan(f32IntegGainQ)
      |       if ~strcmp(f32IntegGainQ_bkup,'0')
      |         set_param(gcb,'f32IntegGainQ','0');
      |       end
      |     else
      |       tmps=num2str(f32IntegGainQ);
      |       if ~strcmp(f32IntegGainQ_bkup,tmps)
      |         set_param(gcb,'f32IntegGainQ',tmps);
      |       end
      |     end
      |     if isnan(s16PropGainShiftQ)
      |       if ~strcmp(s16PropGainShiftQ_bkup,'0')
      |         set_param(gcb,'s16PropGainShiftQ','0');
      |       end
      |     else
      |       tmps=num2str(s16PropGainShiftQ);
      |       if ~strcmp(s16PropGainShiftQ_bkup,tmps)
      |         set_param(gcb,'s16PropGainShiftQ',tmps);
      |       end
      |     end
      |     if isnan(s16IntegGainShiftQ)
      |       if ~strcmp(s16IntegGainShiftQ_bkup,'0')
      |         set_param(gcb,'s16IntegGainShiftQ','0');
      |       end
      |     else
      |       tmps=num2str(s16IntegGainShiftQ);
      |       if ~strcmp(s16IntegGainShiftQ_bkup,tmps)
      |         set_param(gcb,'s16IntegGainShiftQ',tmps);
      |       end
      |     end
      |     if isnan(f32LowerLimitQ)
      |       if ~strcmp(f32LowerLimitQ_bkup,'0')
      |         set_param(gcb,'f32LowerLimitQ','0');
      |       end
      |     else
      |       tmps=num2str(f32LowerLimitQ);
      |       if ~strcmp(f32LowerLimitQ_bkup,tmps)
      |         set_param(gcb,'f32LowerLimitQ',tmps);
      |       end
      |     end
      |     if isnan(f32UpperLimitQ)
      |       if ~strcmp(f32UpperLimitQ_bkup,'0')
      |         set_param(gcb,'f32UpperLimitQ','0');
      |       end
      |     else
      |       tmps=num2str(f32UpperLimitQ);
      |       if ~strcmp(f32UpperLimitQ_bkup,tmps)
      |         set_param(gcb,'f32UpperLimitQ',tmps);
      |       end
      |     end
      |     if isnan(f32RampUp)
      |       if ~strcmp(f32RampUp_bkup,'0')
      |         set_param(gcb,'f32RampUp','0');
      |       end
      |     else
      |       tmps=num2str(f32RampUp);
      |       if ~strcmp(f32RampUp_bkup,tmps)
      |         set_param(gcb,'f32RampUp',tmps);
      |       end
      |     end
      |     if isnan(f32RampDown)
      |       if ~strcmp(f32RampDown_bkup,'0')
      |         set_param(gcb,'f32RampDown','0');
      |       end
      |     else
      |       tmps=num2str(f32RampDown);
      |       if ~strcmp(f32RampDown_bkup,tmps)
      |         set_param(gcb,'f32RampDown',tmps);
      |       end
      |     end
      |   end
      | end
      mask Callback wf0:
      | autoCalcEn=get_param(gcb,'autoCalcEn');
      | if strcmp(autoCalcEn,'on')
      |   SampleTime=Simulink.data.evalinGlobal(bdroot,get_param(gcb,'SampleTime'));
      |   if (SampleTime==-1)
      |     SampleTime=str2double(get_param(gcb,'SampleTime_1'));
      |   end
      |   u16NSamplesW_bkup=get_param(gcb,'u16NSamplesW');
      |   f32PropGainQ_bkup=get_param(gcb,'f32PropGainQ');
      |   f32IntegGainQ_bkup=get_param(gcb,'f32IntegGainQ');
      |   s16PropGainShiftQ_bkup=get_param(gcb,'s16PropGainShiftQ');
      |   s16IntegGainShiftQ_bkup=get_param(gcb,'s16IntegGainShiftQ');
      |   f32LowerLimitQ_bkup=get_param(gcb,'f32LowerLimitQ');
      |   f32UpperLimitQ_bkup=get_param(gcb,'f32UpperLimitQ');
      |   f32RampUp_bkup=get_param(gcb,'f32RampUp');
      |   f32RampDown_bkup=get_param(gcb,'f32RampDown');
      |   wf0=Simulink.data.evalinGlobal(bdroot,get_param(gcb,'wf0'));
      |   wksi=Simulink.data.evalinGlobal(bdroot,get_param(gcb,'wksi'));
      |   J=Simulink.data.evalinGlobal(bdroot,get_param(gcb,'J'));
      |   Kt=Simulink.data.evalinGlobal(bdroot,get_param(gcb,'Kt'));
      |   lambdaW=Simulink.data.evalinGlobal(bdroot,get_param(gcb,'lambdaW'));
      |   ramprpm=Simulink.data.evalinGlobal(bdroot,get_param(gcb,'ramprpm'));
      |   mechspeed=Simulink.data.evalinGlobal(bdroot,get_param(gcb,'mechspeed'));
      |   polepairs=Simulink.data.evalinGlobal(bdroot,get_param(gcb,'polepairs'));
      |   uscale=Simulink.data.evalinGlobal(bdroot,get_param(gcb,'uscale'));
      |   iscale=Simulink.data.evalinGlobal(bdroot,get_param(gcb,'iscale'));
      |   if (wf0<=0)
      |     warning('Natural frequency f0 must be positive.');
      |   end
      |   if (wksi<=0)
      |     warning('Current loop attenuation must be positive.');
      |   end
      |   if (wksi>1)
      |     warning('Current loop attenuation must not exceed 1.');
      |   end
      |   if (J<=0)
      |     warning('Moment of inertia J must be positive.');
      |   end
      |   if (Kt<=0)
      |     warning('Torque constant Kt must be positive.');
      |   end
      |   if (lambdaW<0)
      |     warning('MA filter smoothing factor must be in the range 0..1.');
      |   end
      |   if (lambdaW>1)
      |     warning('MA filter smoothing factor must be in the range 0..1.');
      |   end
      |   if (mechspeed<=0)
      |     warning('Max. speed must be positive.');
      |   end
      |   if (polepairs<1)
      |     warning('Number of pole pairs must be a natural number (1, 2, 3, ...).');
      |   end
      |   if (round(polepairs)~=polepairs)
      |     warning('Number of pole pairs must be a natural number (1, 2, 3, ...).');
      |   end
      |   if (uscale<=0)
      |     warning('U_max must be positive.');
      |   end
      |   if (iscale<=0)
      |     warning('I_max must be positive.');
      |   end
      |   w0=6.283185307179586*wf0;
      |   pgain=2.0*wksi*w0*J/Kt;
      |   igain=w0*w0*J/Kt;
      |   wmax=polepairs*mechspeed*0.1047197551196598;
      |   kpf=pgain*wmax/iscale;
      |   s16PropGainShiftQ=ceil(log2(abs(kpf)));
      |   if s16PropGainShiftQ<-31
      |     s16PropGainShiftQ=-31;
      |   end
      |   if s16PropGainShiftQ>31
      |     s16PropGainShiftQ=31;
      |     warning(['Parameter s16PropGainShiftQ of ' gcb ' exceeds the fixed-point range.']);
      |   end
      |   f32PropGainQ=round(kpf*2^(-s16PropGainShiftQ)*2^31);
      |   if f32PropGainQ>2^31-1
      |     f32PropGainQ=2^31-1;
      |     warning(['Parameter f32PropGainQ of ' gcb ' exceeds the fixed-point range.']);
      |   end
      |   if f32PropGainQ<-2^31
      |     f32PropGainQ=-2^31;
      |     warning(['Parameter f32PropGainQ of ' gcb ' exceeds the fixed-point range.']);
      |   end
      |   kif=igain*SampleTime*0.5*wmax/iscale;
      |   s16IntegGainShiftQ=ceil(log2(abs(kif)));
      |   if s16IntegGainShiftQ<-31
      |     s16IntegGainShiftQ=-31;
      |   end
      |   if s16IntegGainShiftQ>31
      |     s16IntegGainShiftQ=31;
      |     warning(['Parameter s16IntegGainShiftQ of ' gcb ' exceeds the fixed-point range.']);
      |   end
      |   f32IntegGainQ=round(kif*2^(-s16IntegGainShiftQ)*2^31);
      |   if f32IntegGainQ>2^31-1
      |     f32IntegGainQ=2^31-1;
      |     warning(['Parameter f32IntegGainQ of ' gcb ' exceeds the fixed-point range.']);
      |   end
      |   if f32IntegGainQ<-2^31
      |     f32IntegGainQ=-2^31;
      |     warning(['Parameter f32IntegGainQ of ' gcb ' exceeds the fixed-point range.']);
      |   end
      |   f32LowerLimitQ=-2147483648;
      |   f32UpperLimitQ=2147483647;
      |   u16NSamplesW=round(log2(1.0/abs(lambdaW)));
      |   if u16NSamplesW>31
      |     u16NSamplesW=31;
      |   end
      |   if u16NSamplesW<0
      |     u16NSamplesW=0;
      |   end
      |   rampsc=polepairs*abs(ramprpm)*0.1047197551196598/wmax;
      |   f32RampUp=round(rampsc*2^31);
      |   if f32RampUp>2^31-1
      |     f32RampUp=2^31-1;
      |     warning(['Parameter f32RampUp of ' gcb ' exceeds the fixed-point range.']);
      |   end
      |   if f32RampUp<-2^31
      |     f32RampUp=-2^31;
      |     warning(['Parameter f32RampUp of ' gcb ' exceeds the fixed-point range.']);
      |   end
      |   f32RampDown=round(rampsc*2^31);
      |   if f32RampDown>2^31-1
      |     f32RampDown=2^31-1;
      |     warning(['Parameter f32RampDown of ' gcb ' exceeds the fixed-point range.']);
      |   end
      |   if f32RampDown<-2^31
      |     f32RampDown=-2^31;
      |     warning(['Parameter f32RampDown of ' gcb ' exceeds the fixed-point range.']);
      |   end
      |   if isnan(u16NSamplesW)
      |     if ~strcmp(u16NSamplesW_bkup,'0')
      |       set_param(gcb,'u16NSamplesW','0');
      |     end
      |   else
      |     tmps=num2str(u16NSamplesW);
      |     if ~strcmp(u16NSamplesW_bkup,tmps)
      |       set_param(gcb,'u16NSamplesW',tmps);
      |     end
      |   end
      |   if isnan(f32PropGainQ)
      |     if ~strcmp(f32PropGainQ_bkup,'0')
      |       set_param(gcb,'f32PropGainQ','0');
      |     end
      |   else
      |     tmps=num2str(f32PropGainQ);
      |     if ~strcmp(f32PropGainQ_bkup,tmps)
      |       set_param(gcb,'f32PropGainQ',tmps);
      |     end
      |   end
      |   if isnan(f32IntegGainQ)
      |     if ~strcmp(f32IntegGainQ_bkup,'0')
      |       set_param(gcb,'f32IntegGainQ','0');
      |     end
      |   else
      |     tmps=num2str(f32IntegGainQ);
      |     if ~strcmp(f32IntegGainQ_bkup,tmps)
      |       set_param(gcb,'f32IntegGainQ',tmps);
      |     end
      |   end
      |   if isnan(s16PropGainShiftQ)
      |     if ~strcmp(s16PropGainShiftQ_bkup,'0')
      |       set_param(gcb,'s16PropGainShiftQ','0');
      |     end
      |   else
      |     tmps=num2str(s16PropGainShiftQ);
      |     if ~strcmp(s16PropGainShiftQ_bkup,tmps)
      |       set_param(gcb,'s16PropGainShiftQ',tmps);
      |     end
      |   end
      |   if isnan(s16IntegGainShiftQ)
      |     if ~strcmp(s16IntegGainShiftQ_bkup,'0')
      |       set_param(gcb,'s16IntegGainShiftQ','0');
      |     end
      |   else
      |     tmps=num2str(s16IntegGainShiftQ);
      |     if ~strcmp(s16IntegGainShiftQ_bkup,tmps)
